simulink model "ForwardKinematic_YuMi"  (R2024a)
(part 13 of 23)

(7514214926474921*sin(q2L)*((4872700232219253*cos(q1L))/9007199254740992 + (6283307137322267*sin(q1L))/9007199254740992))/36893488147419103232))/1152921504606846976 - (67682029681889335677290557259385*cos(q3L)*((7514214926474921*cos(q2L)*((4872700232219253*cos(q1L))/9007199254740992 + (6283307137322267*sin(q1L))/9007199254740992))/36893488147419103232 - sin(q2L)*((6283307137322267*cos(q1L))/9007199254740992 - (4872700232219253*sin(q1L))/9007199254740992)))/332306998946228968225951765070086144))/9007199254740992 - (7514214926474921*sin(q5L)*(((234819211581865*cos(q4L))/1152921504606846976 + (9007199067919185*sin(q4L))/9007199254740992)*((329794241748012540206902858004467560228111939405*cos(q1L))/2993155353253689176481146537402947624255349848014848 + (425266980168672787164801917791314326747055225795*sin(q1L))/2993155353253689176481146537402947624255349848014848 - (67682029681889335677290557259385*cos(q2L)*((4872700232219253*cos(q1L))/9007199254740992 + (6283307137322267*sin(q1L))/9007199254740992))/332306998946228968225951765070086144 + (9007199067919185*sin(q2L)*((6283307137322267*cos(q1L))/9007199254740992 - (4872700232219253*sin(q1L))/9007199254740992))/9007199254740992) + ((4503599440548691*cos(q4L))/4503599627370496 - (7514214926474921*sin(q4L))/36893488147419103232)*((7514214926474921*sin(q3L)*((7514214926474921*cos(q2L)*((4872700232219253*cos(q1L))/9007199254740992 + (6283307137322267*sin(q1L))/9007199254740992))/36893488147419103232 - sin(q2L)*((6283307137322267*cos(q1L))/9007199254740992 - (4872700232219253*sin(q1L))/9007199254740992)))/36893488147419103232 + (9007199067919185*sin(q3L)*((43889380989894851923989405068805*cos(q1L))/81129638414606681695789005144064 + (56594998190739085871744456992395*sin(q1L))/81129638414606681695789005144064))/9007199254740992 - cos(q3L)*(cos(q2L)*((6283307137322267*cos(q1L))/9007199254740992 - (4872700232219253*sin(q1L))/9007199254740992) + (7514214926474921*sin(q2L)*((4872700232219253*cos(q1L))/9007199254740992 + (6283307137322267*sin(q1L))/9007199254740992))/36893488147419103232)) + (7514214926474921*cos(q4L)*(sin(q3L)*(cos(q2L)*((6283307137322267*cos(q1L))/9007199254740992 - (4872700232219253*sin(q1L))/9007199254740992) + (7514214926474921*sin(q2L)*((4872700232219253*cos(q1L))/9007199254740992 + (6283307137322267*sin(q1L))/9007199254740992))/36893488147419103232) + (9007199067919185*cos(q3L)*((43889380989894851923989405068805*cos(q1L))/81129638414606681695789005144064 + (56594998190739085871744456992395*sin(q1L))/81129638414606681695789005144064))/9007199254740992 + (7514214926474921*cos(q3L)*((7514214926474921*cos(q2L)*((4872700232219253*cos(q1L))/9007199254740992 + (6283307137322267*sin(q1L))/9007199254740992))/36893488147419103232 - sin(q2L)*((6283307137322267*cos(q1L))/9007199254740992 - (4872700232219253*sin(q1L))/9007199254740992)))/36893488147419103232))/36893488147419103232))/36893488147419103232 + cos(q5L)*(((7514214926474921*cos(q4L))/36893488147419103232 + (4503599440548691*sin(q4L))/4503599627370496)*((7514214926474921*sin(q3L)*((7514214926474921*cos(q2L)*((4872700232219253*cos(q1L))/9007199254740992 + (6283307137322267*sin(q1L))/9007199254740992))/36893488147419103232 - sin(q2L)*((6283307137322267*cos(q1L))/9007199254740992 - (4872700232219253*sin(q1L))/9007199254740992)))/36893488147419103232 + (9007199067919185*sin(q3L)*((43889380989894851923989405068805*cos(q1L))/81129638414606681695789005144064 + (56594998190739085871744456992395*sin(q1L))/81129638414606681695789005144064))/9007199254740992 - cos(q3L)*(cos(q2L)*((6283307137322267*cos(q1L))/9007199254740992 - (4872700232219253*sin(q1L))/9007199254740992) + (7514214926474921*sin(q2L)*((4872700232219253*cos(q1L))/9007199254740992 + (6283307137322267*sin(q1L))/9007199254740992))/36893488147419103232)) - ((9007199067919185*cos(q4L))/9007199254740992 - (234819211581865*sin(q4L))/1152921504606846976)*((329794241748012540206902858004467560228111939405*cos(q1L))/2993155353253689176481146537402947624255349848014848 + (425266980168672787164801917791314326747055225795*sin(q1L))/2993155353253689176481146537402947624255349848014848 - (67682029681889335677290557259385*cos(q2L)*((4872700232219253*cos(q1L))/9007199254740992 + (6283307137322267*sin(q1L))/9007199254740992))/332306998946228968225951765070086144 + (9007199067919185*sin(q2L)*((6283307137322267*cos(q1L))/9007199254740992 - (4872700232219253*sin(q1L))/9007199254740992))/9007199254740992) + (7514214926474921*sin(q4L)*(sin(q3L)*(cos(q2L)*((6283307137322267*cos(q1L))/9007199254740992 - (4872700232219253*sin(q1L))/9007199254740992) + (7514214926474921*sin(q2L)*((4872700232219253*cos(q1L))/9007199254740992 + (6283307137322267*sin(q1L))/9007199254740992))/36893488147419103232) + (9007199067919185*cos(q3L)*((43889380989894851923989405068805*cos(q1L))/81129638414606681695789005144064 + (56594998190739085871744456992395*sin(q1L))/81129638414606681695789005144064))/9007199254740992 + (7514214926474921*cos(q3L)*((7514214926474921*cos(q2L)*((4872700232219253*cos(q1L))/9007199254740992 + (6283307137322267*sin(q1L))/9007199254740992))/36893488147419103232 - sin(q2L)*((6283307137322267*cos(q1L))/9007199254740992 - (4872700232219253*sin(q1L))/9007199254740992)))/36893488147419103232))/36893488147419103232)))/1000 + (202883803014822867*sin(q6L)*((7514214926474921*cos(q5L)*(((234819211581865*cos(q4L))/1152921504606846976 + (9007199067919185*sin(q4L))/9007199254740992)*((329794241748012540206902858004467560228111939405*cos(q1L))/2993155353253689176481146537402947624255349848014848 + (425266980168672787164801917791314326747055225795*sin(q1L))/2993155353253689176481146537402947624255349848014848 - (67682029681889335677290557259385*cos(q2L)*((4872700232219253*cos(q1L))/9007199254740992 + (6283307137322267*sin(q1L))/9007199254740992))/332306998946228968225951765070086144 + (9007199067919185*sin(q2L)*((6283307137322267*cos(q1L))/9007199254740992 - (4872700232219253*sin(q1L))/9007199254740992))/9007199254740992) + ((4503599440548691*cos(q4L))/4503599627370496 - (7514214926474921*sin(q4L))/36893488147419103232)*((7514214926474921*sin(q3L)*((7514214926474921*cos(q2L)*((4872700232219253*cos(q1L))/9007199254740992 + (6283307137322267*sin(q1L))/9007199254740992))/36893488147419103232 - sin(q2L)*((6283307137322267*cos(q1L))/9007199254740992 - (4872700232219253*sin(q1L))/9007199254740992)))/36893488147419103232 + (9007199067919185*sin(q3L)*((43889380989894851923989405068805*cos(q1L))/81129638414606681695789005144064 + (56594998190739085871744456992395*sin(q1L))/81129638414606681695789005144064))/9007199254740992 - cos(q3L)*(cos(q2L)*((6283307137322267*cos(q1L))/9007199254740992 - (4872700232219253*sin(q1L))/9007199254740992) + (7514214926474921*sin(q2L)*((4872700232219253*cos(q1L))/9007199254740992 + (6283307137322267*sin(q1L))/9007199254740992))/36893488147419103232)) + (7514214926474921*cos(q4L)*(sin(q3L)*(cos(q2L)*((6283307137322267*cos(q1L))/9007199254740992 - (4872700232219253*sin(q1L))/9007199254740992) + (7514214926474921*sin(q2L)*((4872700232219253*cos(q1L))/9007199254740992 + (6283307137322267*sin(q1L))/9007199254740992))/36893488147419103232) + (9007199067919185*cos(q3L)*((43889380989894851923989405068805*cos(q1L))/81129638414606681695789005144064 + (56594998190739085871744456992395*sin(q1L))/81129638414606681695789005144064))/9007199254740992 + (7514214926474921*cos(q3L)*((7514214926474921*cos(q2L)*((4872700232219253*cos(q1L))/9007199254740992 + (6283307137322267*sin(q1L))/9007199254740992))/36893488147419103232 - sin(q2L)*((6283307137322267*cos(q1L))/9007199254740992 - (4872700232219253*sin(q1L))/9007199254740992)))/36893488147419103232))/36893488147419103232))/36893488147419103232 - (9007199067919185*cos(q5L)*((516845254133432670685844229576986303733782399690601453662320875*cos(q1L))/113078212145816597093331040047546785012958969400039613319782796882727665664 + (666467732349846997487583938718911583194406904318712922873589125*sin(q1L))/113078212145816597093331040047546785012958969400039613319782796882727665664 - (9007199067919185*sin(q3L)*(cos(q2L)*((6283307137322267*cos(q1L))/9007199254740992 - (4872700232219253*sin(q1L))/9007199254740992) + (7514214926474921*sin(q2L)*((4872700232219253*cos(q1L))/9007199254740992 + (6283307137322267*sin(q1L))/9007199254740992))/36893488147419103232))/9007199254740992 + (1764482024691522628700660907665*sin(q3L)*((7514214926474921*cos(q2L)*((4872700232219253*cos(q1L))/9007199254740992 + (6283307137322267*sin(q1L))/9007199254740992))/36893488147419103232 - sin(q2L)*((6283307137322267*cos(q1L))/9007199254740992 - (4872700232219253*sin(q1L))/9007199254740992)))/42535295865117307932921825928971026432 - (106069577339469832923929692356850887620017617375*cos(q2L)*((4872700232219253*cos(q1L))/9007199254740992 + (6283307137322267*sin(q1L))/9007199254740992))/12554203470773361527671578846415332832204710888928069025792 + (14115856197532180673579726082375*sin(q2L)*((6283307137322267*cos(q1L))/9007199254740992 - (4872700232219253*sin(q1L))/9007199254740992))/340282366920938463463374607431768211456 - (81129635049124235038645691064225*cos(q3L)*((43889380989894851923989405068805*cos(q1L))/81129638414606681695789005144064 + (56594998190739085871744456992395*sin(q1L))/81129638414606681695789005144064))/81129638414606681695789005144064 + (2115063383689692319117831580025*sin(q3L)*((43889380989894851923989405068805*cos(q1L))/81129638414606681695789005144064 + (56594998190739085871744456992395*sin(q1L))/81129638414606681695789005144064))/10384593717069655257060992658440192 - (234819211581865*cos(q3L)*(cos(q2L)*((6283307137322267*cos(q1L))/9007199254740992 - (4872700232219253*sin(q1L))/9007199254740992) + (7514214926474921*sin(q2L)*((4872700232219253*cos(q1L))/9007199254740992 + (6283307137322267*sin(q1L))/9007199254740992))/36893488147419103232))/1152921504606846976 - (67682029681889335677290557259385*cos(q3L)*((7514214926474921*cos(q2L)*((4872700232219253*cos(q1L))/9007199254740992 + (6283307137322267*sin(q1L))/9007199254740992))/36893488147419103232 - sin(q2L)*((6283307137322267*cos(q1L))/9007199254740992 - (4872700232219253*sin(q1L))/9007199254740992)))/332306998946228968225951765070086144))/9007199254740992 + sin(q5L)*(((7514214926474921*cos(q4L))/36893488147419103232 + (4503599440548691*sin(q4L))/4503599627370496)*((7514214926474921*sin(q3L)*((7514214926474921*cos(q2L)*((4872700232219253*cos(q1L))/9007199254740992 + (6283307137322267*sin(q1L))/9007199254740992))/36893488147419103232 - sin(q2L)*((6283307137322267*cos(q1L))/9007199254740992 - (4872700232219253*sin(q1L))/9007199254740992)))/36893488147419103232 + (9007199067919185*sin(q3L)*((43889380989894851923989405068805*cos(q1L))/81129638414606681695789005144064 + (56594998190739085871744456992395*sin(q1L))/81129638414606681695789005144064))/9007199254740992 - cos(q3L)*(cos(q2L)*((6283307137322267*cos(q1L))/9007199254740992 - (4872700232219253*sin(q1L))/9007199254740992) + (7514214926474921*sin(q2L)*((4872700232219253*cos(q1L))/9007199254740992 + (6283307137322267*sin(q1L))/9007199254740992))/36893488147419103232)) - ((9007199067919185*cos(q4L))/9007199254740992 - (234819211581865*sin(q4L))/1152921504606846976)*((329794241748012540206902858004467560228111939405*cos(q1L))/2993155353253689176481146537402947624255349848014848 + (425266980168672787164801917791314326747055225795*sin(q1L))/2993155353253689176481146537402947624255349848014848 - (67682029681889335677290557259385*cos(q2L)*((4872700232219253*cos(q1L))/9007199254740992 + (6283307137322267*sin(q1L))/9007199254740992))/332306998946228968225951765070086144 + (9007199067919185*sin(q2L)*((6283307137322267*cos(q1L))/9007199254740992 - (4872700232219253*sin(q1L))/9007199254740992))/9007199254740992) + (7514214926474921*sin(q4L)*(sin(q3L)*(cos(q2L)*((6283307137322267*cos(q1L))/9007199254740992 - (4872700232219253*sin(q1L))/9007199254740992) + (7514214926474921*sin(q2L)*((4872700232219253*cos(q1L))/9007199254740992 + (6283307137322267*sin(q1L))/9007199254740992))/36893488147419103232) + (9007199067919185*cos(q3L)*((43889380989894851923989405068805*cos(q1L))/81129638414606681695789005144064 + (56594998190739085871744456992395*sin(q1L))/81129638414606681695789005144064))/9007199254740992 + (7514214926474921*cos(q3L)*((7514214926474921*cos(q2L)*((4872700232219253*cos(q1L))/9007199254740992 + (6283307137322267*sin(q1L))/9007199254740992))/36893488147419103232 - sin(q2L)*((6283307137322267*cos(q1L))/9007199254740992 - (4872700232219253*sin(q1L))/9007199254740992)))/36893488147419103232))/36893488147419103232)))/36893488147419103232000 - (22542644779424763*sin(q2L)*((4872700232219253*cos(q1L))/9007199254740992 + (6283307137322267*sin(q1L))/9007199254740992))/3689348814741910323200 - (107465779053290185796889472867275736954369330186921663479979246519176992895505610212310958309481948671*sin(q2L)*((6283307137322267*cos(q1L))/9007199254740992 - (4872700232219253*sin(q1L))/9007199254740992))/427197407184182016479004341233910422920540904471330553989408321564443945156128110004592417387315200000 - (324259171862923063*sin(q6L)*((9007199067919185*sin(q5L)*((516845254133432670685844229576986303733782399690601453662320875*cos(q1L))/113078212145816597093331040047546785012958969400039613319782796882727665664 + (666467732349846997487583938718911583194406904318712922873589125*sin(q1L))/113078212145816597093331040047546785012958969400039613319782796882727665664 - (9007199067919185*sin(q3L)*(cos(q2L)*((6283307137322267*cos(q1L))/9007199254740992 - (4872700232219253*sin(q1L))/9007199254740992) + (7514214926474921*sin(q2L)*((4872700232219253*cos(q1L))/9007199254740992 + (6283307137322267*sin(q1L))/9007199254740992))/36893488147419103232))/9007199254740992 + (1764482024691522628700660907665*sin(q3L)*((7514214926474921*cos(q2L)*((4872700232219253*cos(q1L))/9007199254740992 + (6283307137322267*sin(q1L))/9007199254740992))/36893488147419103232 - sin(q2L)*((6283307137322267*cos(q1L))/9007199254740992 - (4872700232219253*sin(q1L))/9007199254740992)))/42535295865117307932921825928971026432 - (106069577339469832923929692356850887620017617375*cos(q2L)*((4872700232219253*cos(q1L))/9007199254740992 + (6283307137322267*sin(q1L))/9007199254740992))/12554203470773361527671578846415332832204710888928069025792 + (14115856197532180673579726082375*sin(q2L)*((6283307137322267*cos(q1L))/9007199254740992 - (4872700232219253*sin(q1L))/9007199254740992))/340282366920938463463374607431768211456 - (81129635049124235038645691064225*cos(q3L)*((43889380989894851923989405068805*cos(q1L))/81129638414606681695789005144064 + (56594998190739085871744456992395*sin(q1L))/81129638414606681695789005144064))/81129638414606681695789005144064 + (2115063383689692319117831580025*sin(q3L)*((43889380989894851923989405068805*cos(q1L))/81129638414606681695789005144064 + (56594998190739085871744456992395*sin(q1L))/81129638414606681695789005144064))/10384593717069655257060992658440192 - (234819211581865*cos(q3L)*(cos(q2L)*((6283307137322267*cos(q1L))/9007199254740992 - (4872700232219253*sin(q1L))/9007199254740992) + (7514214926474921*sin(q2L)*((4872700232219253*cos(q1L))/9007199254740992 + (6283307137322267*sin(q1L))/9007199254740992))/36893488147419103232))/1152921504606846976 - (67682029681889335677290557259385*cos(q3L)*((7514214926474921*cos(q2L)*((4872700232219253*cos(q1L))/9007199254740992 + (6283307137322267*sin(q1L))/9007199254740992))/36893488147419103232 - sin(q2L)*((6283307137322267*cos(q1L))/9007199254740992 - (4872700232219253*sin(q1L))/9007199254740992)))/332306998946228968225951765070086144))/9007199254740992 - (7514214926474921*sin(q5L)*(((234819211581865*cos(q4L))/1152921504606846976 + (9007199067919185*sin(q4L))/9007199254740992)*((329794241748012540206902858004467560228111939405*cos(q1L))/2993155353253689176481146537402947624255349848014848 + (425266980168672787164801917791314326747055225795*sin(q1L))/2993155353253689176481146537402947624255349848014848 - (67682029681889335677290557259385*cos(q2L)*((4872700232219253*cos(q1L))/9007199254740992 + (6283307137322267*sin(q1L))/9007199254740992))/332306998946228968225951765070086144 + (9007199067919185*sin(q2L)*((6283307137322267*cos(q1L))/9007199254740992 - (4872700232219253*sin(q1L))/9007199254740992))/9007199254740992) + ((4503599440548691*cos(q4L))/4503599627370496 - (7514214926474921*sin(q4L))/36893488147419103232)*((7514214926474921*sin(q3L)*((7514214926474921*cos(q2L)*((4872700232219253*cos(q1L))/9007199254740992 + (6283307137322267*sin(q1L))/9007199254740992))/36893488147419103232 - sin(q2L)*((6283307137322267*cos(q1L))/9007199254740992 - (4872700232219253*sin(q1L))/9007199254740992)))/36893488147419103232 + (9007199067919185*sin(q3L)*((43889380989894851923989405068805*cos(q1L))/81129638414606681695789005144064 + (56594998190739085871744456992395*sin(q1L))/81129638414606681695789005144064))/9007199254740992 - cos(q3L)*(cos(q2L)*((6283307137322267*cos(q1L))/9007199254740992 - (4872700232219253*sin(q1L))/9007199254740992) + (7514214926474921*sin(q2L)*((4872700232219253*cos(q1L))/9007199254740992 + (6283307137322267*sin(q1L))/9007199254740992))/36893488147419103232)) + (7514214926474921*cos(q4L)*(sin(q3L)*(cos(q2L)*((6283307137322267*cos(q1L))/9007199254740992 - (4872700232219253*sin(q1L))/9007199254740992) + (7514214926474921*sin(q2L)*((4872700232219253*cos(q1L))/9007199254740992 + (6283307137322267*sin(q1L))/9007199254740992))/36893488147419103232) + (9007199067919185*cos(q3L)*((43889380989894851923989405068805*cos(q1L))/81129638414606681695789005144064 + (56594998190739085871744456992395*sin(q1L))/81129638414606681695789005144064))/9007199254740992 + (7514214926474921*cos(q3L)*((7514214926474921*cos(q2L)*((4872700232219253*cos(q1L))/9007199254740992 + (6283307137322267*sin(q1L))/9007199254740992))/36893488147419103232 - sin(q2L)*((6283307137322267*cos(q1L))/9007199254740992 - (4872700232219253*sin(q1L))/9007199254740992)))/36893488147419103232))/36893488147419103232))/36893488147419103232 + cos(q5L)*(((7514214926474921*cos(q4L))/36893488147419103232 + (4503599440548691*sin(q4L))/4503599627370496)*((7514214926474921*sin(q3L)*((7514214926474921*cos(q2L)*((4872700232219253*cos(q1L))/9007199254740992 + (6283307137322267*sin(q1L))/9007199254740992))/36893488147419103232 - sin(q2L)*((6283307137322267*cos(q1L))/9007199254740992 - (4872700232219253*sin(q1L))/9007199254740992)))/36893488147419103232 + (9007199067919185*sin(q3L)*((43889380989894851923989405068805*cos(q1L))/81129638414606681695789005144064 + (56594998190739085871744456992395*sin(q1L))/81129638414606681695789005144064))/9007199254740992 - cos(q3L)*(cos(q2L)*((6283307137322267*cos(q1L))/9007199254740992 - (4872700232219253*sin(q1L))/9007199254740992) + (7514214926474921*sin(q2L)*((4872700232219253*cos(q1L))/9007199254740992 + (6283307137322267*sin(q1L))/9007199254740992))/36893488147419103232)) - ((9007199067919185*cos(q4L))/9007199254740992 - (234819211581865*sin(q4L))/1152921504606846976)*((329794241748012540206902858004467560228111939405*cos(q1L))/2993155353253689176481146537402947624255349848014848 + (425266980168672787164801917791314326747055225795*sin(q1L))/2993155353253689176481146537402947624255349848014848 - (67682029681889335677290557259385*cos(q2L)*((4872700232219253*cos(q1L))/9007199254740992 + (6283307137322267*sin(q1L))/9007199254740992))/332306998946228968225951765070086144 + (9007199067919185*sin(q2L)*((6283307137322267*cos(q1L))/9007199254740992 - (4872700232219253*sin(q1L))/9007199254740992))/9007199254740992) + (7514214926474921*sin(q4L)*(sin(q3L)*(cos(q2L)*((6283307137322267*cos(q1L))/9007199254740992 - (4872700232219253*sin(q1L))/9007199254740992) + (7514214926474921*sin(q2L)*((4872700232219253*cos(q1L))/9007199254740992 + (6283307137322267*sin(q1L))/9007199254740992))/36893488147419103232) + (9007199067919185*cos(q3L)*((43889380989894851923989405068805*cos(q1L))/81129638414606681695789005144064 + (56594998190739085871744456992395*sin(q1L))/81129638414606681695789005144064))/9007199254740992 + (7514214926474921*cos(q3L)*((7514214926474921*cos(q2L)*((4872700232219253*cos(q1L))/9007199254740992 + (6283307137322267*sin(q1L))/9007199254740992))/36893488147419103232 - sin(q2L)*((6283307137322267*cos(q1L))/9007199254740992 - (4872700232219253*sin(q1L))/9007199254740992)))/36893488147419103232))/36893488147419103232)))/9007199254740992000 - (712008244765680093343103025701132101054572137019*cos(q5L)*(((234819211581865*cos(q4L))/1152921504606846976 + (9007199067919185*sin(q4L))/9007199254740992)*((329794241748012540206902858004467560228111939405*cos(q1L))/2993155353253689176481146537402947624255349848014848 + (425266980168672787164801917791314326747055225795*sin(q1L))/2993155353253689176481146537402947624255349848014848 - (67682029681889335677290557259385*cos(q2L)*((4872700232219253*cos(q1L))/9007199254740992 + (6283307137322267*sin(q1L))/9007199254740992))/332306998946228968225951765070086144 + (9007199067919185*sin(q2L)*((6283307137322267*cos(q1L))/9007199254740992 - (4872700232219253*sin(q1L))/9007199254740992))/9007199254740992) + ((4503599440548691*cos(q4L))/4503599627370496 - (7514214926474921*sin(q4L))/36893488147419103232)*((7514214926474921*sin(q3L)*((7514214926474921*cos(q2L)*((4872700232219253*cos(q1L))/9007199254740992 + (6283307137322267*sin(q1L))/9007199254740992))/36893488147419103232 - sin(q2L)*((6283307137322267*cos(q1L))/9007199254740992 - (4872700232219253*sin(q1L))/9007199254740992)))/36893488147419103232 + (9007199067919185*sin(q3L)*((43889380989894851923989405068805*cos(q1L))/81129638414606681695789005144064 + (56594998190739085871744456992395*sin(q1L))/81129638414606681695789005144064))/9007199254740992 - cos(q3L)*(cos(q2L)*((6283307137322267*cos(q1L))/9007199254740992 - (4872700232219253*sin(q1L))/9007199254740992) + (7514214926474921*sin(q2L)*((4872700232219253*cos(q1L))/9007199254740992 + (6283307137322267*sin(q1L))/9007199254740992))/36893488147419103232)) + (7514214926474921*cos(q4L)*(sin(q3L)*(cos(q2L)*((6283307137322267*cos(q1L))/9007199254740992 - (4872700232219253*sin(q1L))/9007199254740992) + (7514214926474921*sin(q2L)*((4872700232219253*cos(q1L))/9007199254740992 + (6283307137322267*sin(q1L))/9007199254740992))/36893488147419103232) + (9007199067919185*cos(q3L)*((43889380989894851923989405068805*cos(q1L))/81129638414606681695789005144064 + (56594998190739085871744456992395*sin(q1L))/81129638414606681695789005144064))/9007199254740992 + (7514214926474921*cos(q3L)*((7514214926474921*cos(q2L)*((4872700232219253*cos(q1L))/9007199254740992 + (6283307137322267*sin(q1L))/9007199254740992))/36893488147419103232 - sin(q2L)*((6283307137322267*cos(q1L))/9007199254740992 - (4872700232219253*sin(q1L))/9007199254740992)))/36893488147419103232))/36893488147419103232))/2451992865385422173373355243440494693789982595493763481600 + (202883803014822867*sin(q5L)*(((234819211581865*cos(q4L))/1152921504606846976 + (9007199067919185*sin(q4L))/9007199254740992)*((329794241748012540206902858004467560228111939405*cos(q1L))/2993155353253689176481146537402947624255349848014848 + (425266980168672787164801917791314326747055225795*sin(q1L))/2993155353253689176481146537402947624255349848014848 - (67682029681889335677290557259385*cos(q2L)*((4872700232219253*cos(q1L))/9007199254740992 + (6283307137322267*sin(q1L))/9007199254740992))/332306998946228968225951765070086144 + (9007199067919185*sin(q2L)*((6283307137322267*cos(q1L))/9007199254740992 - (4872700232219253*sin(q1L))/9007199254740992))/9007199254740992) + ((4503599440548691*cos(q4L))/4503599627370496 - (7514214926474921*sin(q4L))/36893488147419103232)*((7514214926474921*sin(q3L)*((7514214926474921*cos(q2L)*((4872700232219253*cos(q1L))/9007199254740992 + (6283307137322267*sin(q1L))/9007199254740992))/36893488147419103232 - sin(q2L)*((6283307137322267*cos(q1L))/9007199254740992 - (4872700232219253*sin(q1L))/9007199254740992)))/36893488147419103232 + (9007199067919185*sin(q3L)*((43889380989894851923989405068805*cos(q1L))/81129638414606681695789005144064 + (56594998190739085871744456992395*sin(q1L))/81129638414606681695789005144064))/9007199254740992 - cos(q3L)*(cos(q2L)*((6283307137322267*cos(q1L))/9007199254740992 - (4872700232219253*sin(q1L))/9007199254740992) + (7514214926474921*sin(q2L)*((4872700232219253*cos(q1L))/9007199254740992 + (6283307137322267*sin(q1L))/9007199254740992))/36893488147419103232)) + (7514214926474921*cos(q4L)*(sin(q3L)*(cos(q2L)*((6283307137322267*cos(q1L))/9007199254740992 - (4872700232219253*sin(q1L))/9007199254740992) + (7514214926474921*sin(q2L)*((4872700232219253*cos(q1L))/9007199254740992 + (6283307137322267*sin(q1L))/9007199254740992))/36893488147419103232) + (9007199067919185*cos(q3L)*((43889380989894851923989405068805*cos(q1L))/81129638414606681695789005144064 + (56594998190739085871744456992395*sin(q1L))/81129638414606681695789005144064))/9007199254740992 + (7514214926474921*cos(q3L)*((7514214926474921*cos(q2L)*((4872700232219253*cos(q1L))/9007199254740992 + (6283307137322267*sin(q1L))/9007199254740992))/36893488147419103232 - sin(q2L)*((6283307137322267*cos(q1L))/9007199254740992 - (4872700232219253*sin(q1L))/9007199254740992)))/36893488147419103232))/36893488147419103232))/36893488147419103232000 - (27*cos(q5L)*(((7514214926474921*cos(q4L))/36893488147419103232 + (4503599440548691*sin(q4L))/4503599627370496)*((7514214926474921*sin(q3L)*((7514214926474921*cos(q2L)*((4872700232219253*cos(q1L))/9007199254740992 + (6283307137322267*sin(q1L))/9007199254740992))/36893488147419103232 - sin(q2L)*((6283307137322267*cos(q1L))/9007199254740992 - (4872700232219253*sin(q1L))/9007199254740992)))/36893488147419103232 + (9007199067919185*sin(q3L)*((43889380989894851923989405068805*cos(q1L))/81129638414606681695789005144064 + (56594998190739085871744456992395*sin(q1L))/81129638414606681695789005144064))/9007199254740992 - cos(q3L)*(cos(q2L)*((6283307137322267*cos(q1L))/9007199254740992 - (4872700232219253*sin(q1L))/9007199254740992) + (7514214926474921*sin(q2L)*((4872700232219253*cos(q1L))/9007199254740992 + (6283307137322267*sin(q1L))/9007199254740992))/36893488147419103232)) - ((9007199067919185*cos(q4L))/9007199254740992 - (234819211581865*sin(q4L))/1152921504606846976)*((329794241748012540206902858004467560228111939405*cos(q1L))/2993155353253689176481146537402947624255349848014848 + (425266980168672787164801917791314326747055225795*sin(q1L))/2993155353253689176481146537402947624255349848014848 - (67682029681889335677290557259385*cos(q2L)*((4872700232219253*cos(q1L))/9007199254740992 + (6283307137322267*sin(q1L))/9007199254740992))/332306998946228968225951765070086144 + (9007199067919185*sin(q2L)*((6283307137322267*cos(q1L))/9007199254740992 - (4872700232219253*sin(q1L))/9007199254740992))/9007199254740992) + (7514214926474921*sin(q4L)*(sin(q3L)*(cos(q2L)*((6283307137322267*cos(q1L))/9007199254740992 - (4872700232219253*sin(q1L))/9007199254740992) + (7514214926474921*sin(q2L)*((4872700232219253*cos(q1L))/9007199254740992 + (6283307137322267*sin(q1L))/9007199254740992))/36893488147419103232) + (9007199067919185*cos(q3L)*((43889380989894851923989405068805*cos(q1L))/81129638414606681695789005144064 + (56594998190739085871744456992395*sin(q1L))/81129638414606681695789005144064))/9007199254740992 + (7514214926474921*cos(q3L)*((7514214926474921*cos(q2L)*((4872700232219253*cos(q1L))/9007199254740992 + (6283307137322267*sin(q1L))/9007199254740992))/36893488147419103232 - sin(q2L)*((6283307137322267*cos(q1L))/9007199254740992 - (4872700232219253*sin(q1L))/9007199254740992)))/36893488147419103232))/36893488147419103232))/1000 - (94754841554645069948206780163139*sin(q5L)*(((7514214926474921*cos(q4L))/36893488147419103232 + (4503599440548691*sin(q4L))/4503599627370496)*((7514214926474921*sin(q3L)*((7514214926474921*cos(q2L)*((4872700232219253*cos(q1L))/9007199254740992 + (6283307137322267*sin(q1L))/9007199254740992))/36893488147419103232 - sin(q2L)*((6283307137322267*cos(q1L))/9007199254740992 - (4872700232219253*sin(q1L))/9007199254740992)))/36893488147419103232 + (9007199067919185*sin(q3L)*((43889380989894851923989405068805*cos(q1L))/81129638414606681695789005144064 + (56594998190739085871744456992395*sin(q1L))/81129638414606681695789005144064))/9007199254740992 - cos(q3L)*(cos(q2L)*((6283307137322267*cos(q1L))/9007199254740992 - (4872700232219253*sin(q1L))/9007199254740992) + (7514214926474921*sin(q2L)*((4872700232219253*cos(q1L))/9007199254740992 + (6283307137322267*sin(q1L))/9007199254740992))/36893488147419103232)) - ((9007199067919185*cos(q4L))/9007199254740992 - (234819211581865*sin(q4L))/1152921504606846976)*((329794241748012540206902858004467560228111939405*cos(q1L))/2993155353253689176481146537402947624255349848014848 + (425266980168672787164801917791314326747055225795*sin(q1L))/2993155353253689176481146537402947624255349848014848 - (67682029681889335677290557259385*cos(q2L)*((4872700232219253*cos(q1L))/9007199254740992 + (6283307137322267*sin(q1L))/9007199254740992))/332306998946228968225951765070086144 + (9007199067919185*sin(q2L)*((6283307137322267*cos(q1L))/9007199254740992 - (4872700232219253*sin(q1L))/9007199254740992))/9007199254740992) + (7514214926474921*sin(q4L)*(sin(q3L)*(cos(q2L)*((6283307137322267*cos(q1L))/9007199254740992 - (4872700232219253*sin(q1L))/9007199254740992) + (7514214926474921*sin(q2L)*((4872700232219253*cos(q1L))/9007199254740992 + (6283307137322267*sin(q1L))/9007199254740992))/36893488147419103232) + (9007199067919185*cos(q3L)*((43889380989894851923989405068805*cos(q1L))/81129638414606681695789005144064 + (56594998190739085871744456992395*sin(q1L))/81129638414606681695789005144064))/9007199254740992 + (7514214926474921*cos(q3L)*((7514214926474921*cos(q2L)*((4872700232219253*cos(q1L))/9007199254740992 + (6283307137322267*sin(q1L))/9007199254740992))/36893488147419103232 - sin(q2L)*((6283307137322267*cos(q1L))/9007199254740992 - (4872700232219253*sin(q1L))/9007199254740992)))/36893488147419103232))/36893488147419103232))/66461399789245793645190353014017228800 - (83301539375654672537075965313343183841442266989297270401707771044036658496661398777306991*cos(q3L)*((43889380989894851923989405068805*cos(q1L))/81129638414606681695789005144064 + (56594998190739085871744456992395*sin(q1L))/81129638414606681695789005144064))/4074071952668972172536891376818756322102936787331872501272280898708762599526673412366794752000 + (610321541873521657855151997354401418608858870661075444886782706002880706727*cos(q4L)*(sin(q3L)*(cos(q2L)*((6283307137322267*cos(q1L))/9007199254740992 - (4872700232219253*sin(q1L))/9007199254740992) + (7514214926474921*sin(q2L)*((4872700232219253*cos(q1L))/9007199254740992 + (6283307137322267*sin(q1L))/9007199254740992))/36893488147419103232) + (9007199067919185*cos(q3L)*((43889380989894851923989405068805*cos(q1L))/81129638414606681695789005144064 + (56594998190739085871744456992395*sin(q1L))/81129638414606681695789005144064))/9007199254740992 + (7514214926474921*cos(q3L)*((7514214926474921*cos(q2L)*((4872700232219253*cos(q1L))/9007199254740992 + (6283307137322267*sin(q1L))/9007199254740992))/36893488147419103232 - sin(q2L)*((6283307137322267*cos(q1L))/9007199254740992 - (4872700232219253*sin(q1L))/9007199254740992)))/36893488147419103232))/11307821214581659709333104004754678501295896940003961331978279688272766566400000 + (109198173955282063961996941994332957526645881091499469714283881779231664456243735535448036415347*sin(q3L)*((43889380989894851923989405068805*cos(q1L))/81129638414606681695789005144064 + (56594998190739085871744456992395*sin(q1L))/81129638414606681695789005144064))/2607406049708142190423610481164004046145879543892398400814259775173608063697070983914748641280000 + (608651409044468601*sin(q4L)*(sin(q3L)*(cos(q2L)*((6283307137322267*cos(q1L))/9007199254740992 - (4872700232219253*sin(q1L))/9007199254740992) + (7514214926474921*sin(q2L)*((4872700232219253*cos(q1L))/9007199254740992 + (6283307137322267*sin(q1L))/9007199254740992))/36893488147419103232) + (9007199067919185*cos(q3L)*((43889380989894851923989405068805*cos(q1L))/81129638414606681695789005144064 + (56594998190739085871744456992395*sin(q1L))/81129638414606681695789005144064))/9007199254740992 + (7514214926474921*cos(q3L)*((7514214926474921*cos(q2L)*((4872700232219253*cos(q1L))/9007199254740992 + (6283307137322267*sin(q1L))/9007199254740992))/36893488147419103232 - sin(q2L)*((6283307137322267*cos(q1L))/9007199254740992 - (4872700232219253*sin(q1L))/9007199254740992)))/36893488147419103232))/73786976294838206464000 - (60617164743372705924380750591060836759586313939367162716784907429017787816377231*cos(q3L)*(cos(q2L)*((6283307137322267*cos(q1L))/9007199254740992 - (4872700232219253*sin(q1L))/9007199254740992) + (7514214926474921*sin(q2L)*((4872700232219253*cos(q1L))/9007199254740992 + (6283307137322267*sin(q1L))/9007199254740992))/36893488147419103232))/1447401115466452442794637312608598848165874808320507050493219800098914120499200000 - (347469655025336708709976918716104493695816557877713443586884917071777956519687017125887603*cos(q3L)*((7514214926474921*cos(q2L)*((4872700232219253*cos(q1L))/9007199254740992 + (6283307137322267*sin(q1L))/9007199254740992))/36893488147419103232 - sin(q2L)*((6283307137322267*cos(q1L))/9007199254740992 - (4872700232219253*sin(q1L))/9007199254740992)))/83436993590660550093555535397248129476668145404556748826056312805555458038306271485271956520960000, (324259171862923063*sin(q6L)*((7514214926474921*sin(q5L)*(((4503599440548691*cos(q4L))/4503599627370496 - (7514214926474921*sin(q4L))/36893488147419103232)*(cos(q3L)*((7514214926474921*cos(q2L)*((6283307137322267*cos(q1L))/9007199254740992 - (4872700232219253*sin(q1L))/9007199254740992))/36893488147419103232 - (76229820211215127867025072518845*cos(q2L))/162259276829213363391578010288128 + sin(q2L)*((4872700232219253*cos(q1L))/9007199254740992 + (6283307137322267*sin(q1L))/9007199254740992)) - (7514214926474921*sin(q3L)*((76229820211215127867025072518845*sin(q2L))/162259276829213363391578010288128 + cos(q2L)*((4872700232219253*cos(q1L))/9007199254740992 + (6283307137322267*sin(q1L))/9007199254740992) - (7514214926474921*sin(q2L)*((6283307137322267*cos(q1L))/9007199254740992 - (4872700232219253*sin(q1L))/9007199254740992))/36893488147419103232))/36893488147419103232) + ((234819211581865*cos(q4L))/1152921504606846976 + (9007199067919185*sin(q4L))/9007199254740992)*((686617165554103949950999710565799465200849541325*sin(q2L))/1461501637330902918203684832716283019655932542976 + (9007199067919185*cos(q2L)*((4872700232219253*cos(q1L))/9007199254740992 + (6283307137322267*sin(q1L))/9007199254740992))/9007199254740992 - (67682029681889335677290557259385*sin(q2L)*((6283307137322267*cos(q1L))/9007199254740992 - (4872700232219253*sin(q1L))/9007199254740992))/332306998946228968225951765070086144) - (7514214926474921*cos(q4L)*((7514214926474921*cos(q3L)*((76229820211215127867025072518845*sin(q2L))/162259276829213363391578010288128 + cos(q2L)*((4872700232219253*cos(q1L))/9007199254740992 + (6283307137322267*sin(q1L))/9007199254740992) - (7514214926474921*sin(q2L)*((6283307137322267*cos(q1L))/9007199254740992 - (4872700232219253*sin(q1L))/9007199254740992))/36893488147419103232))/36893488147419103232 + sin(q3L)*((7514214926474921*cos(q2L)*((6283307137322267*cos(q1L))/9007199254740992 - (4872700232219253*sin(q1L))/9007199254740992))/36893488147419103232 - (76229820211215127867025072518845*cos(q2L))/162259276829213363391578010288128 + sin(q2L)*((4872700232219253*cos(q1L))/9007199254740992 + (6283307137322267*sin(q1L))/9007199254740992))))/36893488147419103232))/36893488147419103232 + cos(q5L)*(((9007199067919185*cos(q4L))/9007199254740992 - (234819211581865*sin(q4L))/1152921504606846976)*((686617165554103949950999710565799465200849541325*sin(q2L))/1461501637330902918203684832716283019655932542976 + (9007199067919185*cos(q2L)*((4872700232219253*cos(q1L))/9007199254740992 + (6283307137322267*sin(q1L))/9007199254740992))/9007199254740992 - (67682029681889335677290557259385*sin(q2L)*((6283307137322267*cos(q1L))/9007199254740992 - (4872700232219253*sin(q1L))/9007199254740992))/332306998946228968225951765070086144) - ((7514214926474921*cos(q4L))/36893488147419103232 + (4503599440548691*sin(q4L))/4503599627370496)*(cos(q3L)*((7514214926474921*cos(q2L)*((6283307137322267*cos(q1L))/9007199254740992 - (4872700232219253*sin(q1L))/9007199254740992))/36893488147419103232 - (76229820211215127867025072518845*cos(q2L))/162259276829213363391578010288128 + sin(q2L)*((4872700232219253*cos(q1L))/9007199254740992 + (6283307137322267*sin(q1L))/9007199254740992)) - (7514214926474921*sin(q3L)*((76229820211215127867025072518845*sin(q2L))/162259276829213363391578010288128 + cos(q2L)*((4872700232219253*cos(q1L))/9007199254740992 + (6283307137322267*sin(q1L))/9007199254740992) - (7514214926474921*sin(q2L)*((6283307137322267*cos(q1L))/9007199254740992 - (4872700232219253*sin(q1L))/9007199254740992))/36893488147419103232))/36893488147419103232) + (7514214926474921*sin(q4L)*((7514214926474921*cos(q3L)*((76229820211215127867025072518845*sin(q2L))/162259276829213363391578010288128 + cos(q2L)*((4872700232219253*cos(q1L))/9007199254740992 + (6283307137322267*sin(q1L))/9007199254740992) - (7514214926474921*sin(q2L)*((6283307137322267*cos(q1L))/9007199254740992 - (4872700232219253*sin(q1L))/9007199254740992))/36893488147419103232))/36893488147419103232 + sin(q3L)*((7514214926474921*cos(q2L)*((6283307137322267*cos(q1L))/9007199254740992 - (4872700232219253*sin(q1L))/9007199254740992))/36893488147419103232 - (76229820211215127867025072518845*cos(q2L))/162259276829213363391578010288128 + sin(q2L)*((4872700232219253*cos(q1L))/9007199254740992 + (6283307137322267*sin(q1L))/9007199254740992))))/36893488147419103232) - (9007199067919185*sin(q5L)*((1076049180065244948668759145796765391250102872519935285209856875*sin(q2L))/55213970774324510299478046898216203619608871777363092441300193790394368 + (234819211581865*cos(q3L)*((7514214926474921*cos(q2L)*((6283307137322267*cos(q1L))/9007199254740992 - (4872700232219253*sin(q1L))/9007199254740992))/36893488147419103232 - (76229820211215127867025072518845*cos(q2L))/162259276829213363391578010288128 + sin(q2L)*((4872700232219253*cos(q1L))/9007199254740992 + (6283307137322267*sin(q1L))/9007199254740992)))/1152921504606846976 + (67682029681889335677290557259385*cos(q3L)*((76229820211215127867025072518845*sin(q2L))/162259276829213363391578010288128 + cos(q2L)*((4872700232219253*cos(q1L))/9007199254740992 + (6283307137322267*sin(q1L))/9007199254740992) - (7514214926474921*sin(q2L)*((6283307137322267*cos(q1L))/9007199254740992 - (4872700232219253*sin(q1L))/9007199254740992))/36893488147419103232))/332306998946228968225951765070086144 + (9007199067919185*sin(q3L)*((7514214926474921*cos(q2L)*((6283307137322267*cos(q1L))/9007199254740992 - (4872700232219253*sin(q1L))/9007199254740992))/36893488147419103232 - (76229820211215127867025072518845*cos(q2L))/162259276829213363391578010288128 + sin(q2L)*((4872700232219253*cos(q1L))/9007199254740992 + (6283307137322267*sin(q1L))/9007199254740992)))/9007199254740992 - (1764482024691522628700660907665*sin(q3L)*((76229820211215127867025072518845*sin(q2L))/162259276829213363391578010288128 + cos(q2L)*((4872700232219253*cos(q1L))/9007199254740992 + (6283307137322267*sin(q1L))/9007199254740992) - (7514214926474921*sin(q2L)*((6283307137322267*cos(q1L))/9007199254740992 - (4872700232219253*sin(q1L))/9007199254740992))/36893488147419103232))/42535295865117307932921825928971026432 + (14115856197532180673579726082375*cos(q2L)*((4872700232219253*cos(q1L))/9007199254740992 + (6283307137322267*sin(q1L))/9007199254740992))/340282366920938463463374607431768211456 - (106069577339469832923929692356850887620017617375*sin(q2L)*((6283307137322267*cos(q1L))/9007199254740992 - (4872700232219253*sin(q1L))/9007199254740992))/12554203470773361527671578846415332832204710888928069025792))/9007199254740992))/9007199254740992000 - (1638419403218095907026718462896803369073888043416845373610358683372970217080019045088391026475339262573991311605362042051448194040999*sin(q2L))/13863348470604074297892070920715418517182185376879082875852397903073106539028128115199872030520697890486956054807017859144870789120000 - (45737892126729076720215043511307*cos(q2L))/3245185536584267267831560205762560 + (81222263116692158804177042061221826384594597321566869716687*((4503599440548691*cos(q4L))/4503599627370496 - (7514214926474921*sin(q4L))/36893488147419103232)*(cos(q3L)*((7514214926474921*cos(q2L)*((6283307137322267*cos(q1L))/9007199254740992 - (4872700232219253*sin(q1L))/9007199254740992))/36893488147419103232 - (76229820211215127867025072518845*cos(q2L))/162259276829213363391578010288128 + sin(q2L)*((4872700232219253*cos(q1L))/9007199254740992 + (6283307137322267*sin(q1L))/9007199254740992)) - (7514214926474921*sin(q3L)*((76229820211215127867025072518845*sin(q2L))/162259276829213363391578010288128 + cos(q2L)*((4872700232219253*cos(q1L))/9007199254740992 + (6283307137322267*sin(q1L))/9007199254740992) - (7514214926474921*sin(q2L)*((6283307137322267*cos(q1L))/9007199254740992 - (4872700232219253*sin(q1L))/9007199254740992))/36893488147419103232))/36893488147419103232))/306499108173177771671669405430061836723747824436720435200000 + (81*((7514214926474921*cos(q4L))/36893488147419103232 + (4503599440548691*sin(q4L))/4503599627370496)*(cos(q3L)*((7514214926474921*cos(q2L)*((6283307137322267*cos(q1L))/9007199254740992 - (4872700232219253*sin(q1L))/9007199254740992))/36893488147419103232 - (76229820211215127867025072518845*cos(q2L))/162259276829213363391578010288128 + sin(q2L)*((4872700232219253*cos(q1L))/9007199254740992 + (6283307137322267*sin(q1L))/9007199254740992)) - (7514214926474921*sin(q3L)*((76229820211215127867025072518845*sin(q2L))/162259276829213363391578010288128 + cos(q2L)*((4872700232219253*cos(q1L))/9007199254740992 + (6283307137322267*sin(q1L))/9007199254740992) - (7514214926474921*sin(q2L)*((6283307137322267*cos(q1L))/9007199254740992 - (4872700232219253*sin(q1L))/9007199254740992))/36893488147419103232))/36893488147419103232))/2000 + (60617164743372705924380750591060836759586313939367162716784907429017787816377231*cos(q3L)*((7514214926474921*cos(q2L)*((6283307137322267*cos(q1L))/9007199254740992 - (4872700232219253*sin(q1L))/9007199254740992))/36893488147419103232 - (76229820211215127867025072518845*cos(q2L))/162259276829213363391578010288128 + sin(q2L)*((4872700232219253*cos(q1L))/9007199254740992 + (6283307137322267*sin(q1L))/9007199254740992)))/1447401115466452442794637312608598848165874808320507050493219800098914120499200000 + (347469655025336708709976918716104493695816557877713443586884917071777956519687017125887603*cos(q3L)*((76229820211215127867025072518845*sin(q2L))/162259276829213363391578010288128 + cos(q2L)*((4872700232219253*cos(q1L))/9007199254740992 + (6283307137322267*sin(q1L))/9007199254740992) - (7514214926474921*sin(q2L)*((6283307137322267*cos(q1L))/9007199254740992 - (4872700232219253*sin(q1L))/9007199254740992))/36893488147419103232))/83436993590660550093555535397248129476668145404556748826056312805555458038306271485271956520960000 + (46241644459901303158631016767207157814229090534989303509431886332469146043*sin(q3L)*((7514214926474921*cos(q2L)*((6283307137322267*cos(q1L))/9007199254740992 - (4872700232219253*sin(q1L))/9007199254740992))/36893488147419103232 - (76229820211215127867025072518845*cos(q2L))/162259276829213363391578010288128 + sin(q2L)*((4872700232219253*cos(q1L))/9007199254740992 + (6283307137322267*sin(q1L))/9007199254740992)))/2261564242916331941866620800950935700259179388000792266395655937654553313280000 - (455490404115240510935077772268745492204390157443214084883134054419271951750419293234291596923751*sin(q3L)*((76229820211215127867025072518845*sin(q2L))/162259276829213363391578010288128 + cos(q2L)*((4872700232219253*cos(q1L))/9007199254740992 + (6283307137322267*sin(q1L))/9007199254740992) - (7514214926474921*sin(q2L)*((6283307137322267*cos(q1L))/9007199254740992 - (4872700232219253*sin(q1L))/9007199254740992))/36893488147419103232))/53399675898022752059875542654238802865067613058916319248676040195555493144516013750574052173414400000 + (584133382113593486367040631332731*cos(q6L)*((8085664810467363599778659999511780427732698420102663058998013758035866686931875*sin(q2L))/2037035976334486086268445688409378161051468393665936250636140449354381299763336706183397376 + (9007199067919185*((4503599440548691*cos(q4L))/4503599627370496 - (7514214926474921*sin(q4L))/36893488147419103232)*(cos(q3L)*((7514214926474921*cos(q2L)*((6283307137322267*cos(q1L))/9007199254740992 - (4872700232219253*sin(q1L))/9007199254740992))/36893488147419103232 - (76229820211215127867025072518845*cos(q2L))/162259276829213363391578010288128 + sin(q2L)*((4872700232219253*cos(q1L))/9007199254740992 + (6283307137322267*sin(q1L))/9007199254740992)) - (7514214926474921*sin(q3L)*((76229820211215127867025072518845*sin(q2L))/162259276829213363391578010288128 + cos(q2L)*((4872700232219253*cos(q1L))/9007199254740992 + (6283307137322267*sin(q1L))/9007199254740992) - (7514214926474921*sin(q2L)*((6283307137322267*cos(q1L))/9007199254740992 - (4872700232219253*sin(q1L))/9007199254740992))/36893488147419103232))/36893488147419103232))/9007199254740992 + (1764482024691522628700660907665*cos(q3L)*((7514214926474921*cos(q2L)*((6283307137322267*cos(q1L))/9007199254740992 - (4872700232219253*sin(q1L))/9007199254740992))/36893488147419103232 - (76229820211215127867025072518845*cos(q2L))/162259276829213363391578010288128 + sin(q2L)*((4872700232219253*cos(q1L))/9007199254740992 + (6283307137322267*sin(q1L))/9007199254740992)))/42535295865117307932921825928971026432 + (508577317689771495245073589786522929324694383585*cos(q3L)*((76229820211215127867025072518845*sin(q2L))/162259276829213363391578010288128 + cos(q2L)*((4872700232219253*cos(q1L))/9007199254740992 + (6283307137322267*sin(q1L))/9007199254740992) - (7514214926474921*sin(q2L)*((6283307137322267*cos(q1L))/9007199254740992 - (4872700232219253*sin(q1L))/9007199254740992))/36893488147419103232))/12259964326927110866866776217202473468949912977468817408 + (67682029681889335677290557259385*sin(q3L)*((7514214926474921*cos(q2L)*((6283307137322267*cos(q1L))/9007199254740992 - (4872700232219253*sin(q1L))/9007199254740992))/36893488147419103232 - (76229820211215127867025072518845*cos(q2L))/162259276829213363391578010288128 + sin(q2L)*((4872700232219253*cos(q1L))/9007199254740992 + (6283307137322267*sin(q1L))/9007199254740992)))/332306998946228968225951765070086144 - (13258697167433729449897784796786197386719169465*sin(q3L)*((76229820211215127867025072518845*sin(q2L))/162259276829213363391578010288128 + cos(q2L)*((4872700232219253*cos(q1L))/9007199254740992 + (6283307137322267*sin(q1L))/9007199254740992) - (7514214926474921*sin(q2L)*((6283307137322267*cos(q1L))/9007199254740992 - (4872700232219253*sin(q1L))/9007199254740992))/36893488147419103232))/1569275433846670190958947355801916604025588861116008628224 + (106069577339469832923929692356850887620017617375*cos(q2L)*((4872700232219253*cos(q1L))/9007199254740992 + (6283307137322267*sin(q1L))/9007199254740992))/12554203470773361527671578846415332832204710888928069025792 - (797029601289130257223357069404502671534492977261568326111352375*sin(q2L)*((6283307137322267*cos(q1L))/9007199254740992 - (4872700232219253*sin(q1L))/9007199254740992))/463168356949264781694283940034751631413079938662562256157830336031652518559744 + (9007199067919185*((234819211581865*cos(q4L))/1152921504606846976 + (9007199067919185*sin(q4L))/9007199254740992)*((686617165554103949950999710565799465200849541325*sin(q2L))/1461501637330902918203684832716283019655932542976 + (9007199067919185*cos(q2L)*((4872700232219253*cos(q1L))/9007199254740992 + (6283307137322267*sin(q1L))/9007199254740992))/9007199254740992 - (67682029681889335677290557259385*sin(q2L)*((6283307137322267*cos(q1L))/9007199254740992 - (4872700232219253*sin(q1L))/9007199254740992))/332306998946228968225951765070086144))/9007199254740992 - (67682029681889335677290557259385*cos(q4L)*((7514214926474921*cos(q3L)*((76229820211215127867025072518845*sin(q2L))/162259276829213363391578010288128 + cos(q2L)*((4872700232219253*cos(q1L))/9007199254740992 + (6283307137322267*sin(q1L))/9007199254740992) - (7514214926474921*sin(q2L)*((6283307137322267*cos(q1L))/9007199254740992 - (4872700232219253*sin(q1L))/9007199254740992))/36893488147419103232))/36893488147419103232 + sin(q3L)*((7514214926474921*cos(q2L)*((6283307137322267*cos(q1L))/9007199254740992 - (4872700232219253*sin(q1L))/9007199254740992))/36893488147419103232 - (76229820211215127867025072518845*cos(q2L))/162259276829213363391578010288128 + sin(q2L)*((4872700232219253*cos(q1L))/9007199254740992 + (6283307137322267*sin(q1L))/9007199254740992))))/332306998946228968225951765070086144))/16225927682921336339157801028812800 - (107465779053290185796889472867275736954369330186921663479979246519176992895505610212310958309481948671*cos(q2L)*((4872700232219253*cos(q1L))/9007199254740992 + (6283307137322267*sin(q1L))/9007199254740992))/427197407184182016479004341233910422920540904471330553989408321564443945156128110004592417387315200000 + (22542644779424763*cos(q2L)*((6283307137322267*cos(q1L))/9007199254740992 - (4872700232219253*sin(q1L))/9007199254740992))/3689348814741910323200 + (48638874966763599*sin(q6L)*((8085664810467363599778659999511780427732698420102663058998013758035866686931875*sin(q2L))/2037035976334486086268445688409378161051468393665936250636140449354381299763336706183397376 + (9007199067919185*((4503599440548691*cos(q4L))/4503599627370496 - (7514214926474921*sin(q4L))/36893488147419103232)*(cos(q3L)*((7514214926474921*cos(q2L)*((6283307137322267*cos(q1L))/9007199254740992 - (4872700232219253*sin(q1L))/9007199254740992))/36893488147419103232 - (76229820211215127867025072518845*cos(q2L))/162259276829213363391578010288128 + sin(q2L)*((4872700232219253*cos(q1L))/9007199254740992 + (6283307137322267*sin(q1L))/9007199254740992)) - (7514214926474921*sin(q3L)*((76229820211215127867025072518845*sin(q2L))/162259276829213363391578010288128 + cos(q2L)*((4872700232219253*cos(q1L))/9007199254740992 + (6283307137322267*sin(q1L))/9007199254740992) - (7514214926474921*sin(q2L)*((6283307137322267*cos(q1L))/9007199254740992 - (4872700232219253*sin(q1L))/9007199254740992))/36893488147419103232))/36893488147419103232))/9007199254740992 + (1764482024691522628700660907665*cos(q3L)*((7514214926474921*cos(q2L)*((6283307137322267*cos(q1L))/9007199254740992 - (4872700232219253*sin(q1L))/9007199254740992))/36893488147419103232 - (76229820211215127867025072518845*cos(q2L))/162259276829213363391578010288128 + sin(q2L)*((4872700232219253*cos(q1L))/9007199254740992 + (6283307137322267*sin(q1L))/9007199254740992)))/42535295865117307932921825928971026432 + (508577317689771495245073589786522929324694383585*cos(q3L)*((76229820211215127867025072518845*sin(q2L))/162259276829213363391578010288128 + cos(q2L)*((4872700232219253*cos(q1L))/9007199254740992 + (6283307137322267*sin(q1L))/9007199254740992) - (7514214926474921*sin(q2L)*((6283307137322267*cos(q1L))/9007199254740992 - (4872700232219253*sin(q1L))/9007199254740992))/36893488147419103232))/12259964326927110866866776217202473468949912977468817408 + (67682029681889335677290557259385*sin(q3L)*((7514214926474921*cos(q2L)*((6283307137322267*cos(q1L))/9007199254740992 - (4872700232219253*sin(q1L))/9007199254740992))/36893488147419103232 - (76229820211215127867025072518845*cos(q2L))/162259276829213363391578010288128 + sin(q2L)*((4872700232219253*cos(q1L))/9007199254740992 + (6283307137322267*sin(q1L))/9007199254740992)))/332306998946228968225951765070086144 - (13258697167433729449897784796786197386719169465*sin(q3L)*((76229820211215127867025072518845*sin(q2L))/162259276829213363391578010288128 + cos(q2L)*((4872700232219253*cos(q1L))/9007199254740992 + (6283307137322267*sin(q1L))/9007199254740992) - (7514214926474921*sin(q2L)*((6283307137322267*cos(q1L))/9007199254740992 - (4872700232219253*sin(q1L))/9007199254740992))/36893488147419103232))/1569275433846670190958947355801916604025588861116008628224 + (106069577339469832923929692356850887620017617375*cos(q2L)*((4872700232219253*cos(q1L))/9007199254740992 + (6283307137322267*sin(q1L))/9007199254740992))/12554203470773361527671578846415332832204710888928069025792 - (797029601289130257223357069404502671534492977261568326111352375*sin(q2L)*((6283307137322267*cos(q1L))/9007199254740992 - (4872700232219253*sin(q1L))/9007199254740992))/463168356949264781694283940034751631413079938662562256157830336031652518559744 + (9007199067919185*((234819211581865*cos(q4L))/1152921504606846976 + (9007199067919185*sin(q4L))/9007199254740992)*((686617165554103949950999710565799465200849541325*sin(q2L))/1461501637330902918203684832716283019655932542976 + (9007199067919185*cos(q2L)*((4872700232219253*cos(q1L))/9007199254740992 + (6283307137322267*sin(q1L))/9007199254740992))/9007199254740992 - (67682029681889335677290557259385*sin(q2L)*((6283307137322267*cos(q1L))/9007199254740992 - (4872700232219253*sin(q1L))/9007199254740992))/332306998946228968225951765070086144))/9007199254740992 - (67682029681889335677290557259385*cos(q4L)*((7514214926474921*cos(q3L)*((76229820211215127867025072518845*sin(q2L))/162259276829213363391578010288128 + cos(q2L)*((4872700232219253*cos(q1L))/9007199254740992 + (6283307137322267*sin(q1L))/9007199254740992) - (7514214926474921*sin(q2L)*((6283307137322267*cos(q1L))/9007199254740992 - (4872700232219253*sin(q1L))/9007199254740992))/36893488147419103232))/36893488147419103232 + sin(q3L)*((7514214926474921*cos(q2L)*((6283307137322267*cos(q1L))/9007199254740992 - (4872700232219253*sin(q1L))/9007199254740992))/36893488147419103232 - (76229820211215127867025072518845*cos(q2L))/162259276829213363391578010288128 + sin(q2L)*((4872700232219253*cos(q1L))/9007199254740992 + (6283307137322267*sin(q1L))/9007199254740992))))/332306998946228968225951765070086144))/1801439850948198400 - (712008244765680093343103025701132101054572137019*cos(q5L)*(((4503599440548691*cos(q4L))/4503599627370496 - (7514214926474921*sin(q4L))/36893488147419103232)*(cos(q3L)*((7514214926474921*cos(q2L)*((6283307137322267*cos(q1L))/9007199254740992 - (4872700232219253*sin(q1L))/9007199254740992))/36893488147419103232 - (76229820211215127867025072518845*cos(q2L))/162259276829213363391578010288128 + sin(q2L)*((4872700232219253*cos(q1L))/9007199254740992 + (6283307137322267*sin(q1L))/9007199254740992)) - (7514214926474921*sin(q3L)*((76229820211215127867025072518845*sin(q2L))/162259276829213363391578010288128 + cos(q2L)*((4872700232219253*cos(q1L))/9007199254740992 + (6283307137322267*sin(q1L))/9007199254740992) - (7514214926474921*sin(q2L)*((6283307137322267*cos(q1L))/9007199254740992 - (4872700232219253*sin(q1L))/9007199254740992))/36893488147419103232))/36893488147419103232) + ((234819211581865*cos(q4L))/1152921504606846976 + (9007199067919185*sin(q4L))/9007199254740992)*((686617165554103949950999710565799465200849541325*sin(q2L))/1461501637330902918203684832716283019655932542976 + (9007199067919185*cos(q2L)*((4872700232219253*cos(q1L))/9007199254740992 + (6283307137322267*sin(q1L))/9007199254740992))/9007199254740992 - (67682029681889335677290557259385*sin(q2L)*((6283307137322267*cos(q1L))/9007199254740992 - (4872700232219253*sin(q1L))/9007199254740992))/332306998946228968225951765070086144) - (7514214926474921*cos(q4L)*((7514214926474921*cos(q3L)*((76229820211215127867025072518845*sin(q2L))/162259276829213363391578010288128 + cos(q2L)*((4872700232219253*cos(q1L))/9007199254740992 + (6283307137322267*sin(q1L))/9007199254740992) - (7514214926474921*sin(q2L)*((6283307137322267*cos(q1L))/9007199254740992 - (4872700232219253*sin(q1L))/9007199254740992))/36893488147419103232))/36893488147419103232 + sin(q3L)*((7514214926474921*cos(q2L)*((6283307137322267*cos(q1L))/9007199254740992 - (4872700232219253*sin(q1L))/9007199254740992))/36893488147419103232 - (76229820211215127867025072518845*cos(q2L))/162259276829213363391578010288128 + sin(q2L)*((4872700232219253*cos(q1L))/9007199254740992 + (6283307137322267*sin(q1L))/9007199254740992))))/36893488147419103232))/2451992865385422173373355243440494693789982595493763481600 + (3*sin(q2L)*((4872700232219253*cos(q1L))/9007199254740992 + (6283307137322267*sin(q1L))/9007199254740992))/100 + (807520961047489018778067709720399904923771262077295170375712179706208528987338271217011451790113918662491539890779991*sin(q2L)*((6283307137322267*cos(q1L))/9007199254740992 - (4872700232219253*sin(q1L))/9007199254740992))/15760802478557791684911616040057445522031895708186178667179317361698288708598884244565706501953966256322651196122726400000 + (202883803014822867*sin(q5L)*(((4503599440548691*cos(q4L))/4503599627370496 - (7514214926474921*sin(q4L))/36893488147419103232)*(cos(q3L)*((7514214926474921*cos(q2L)*((6283307137322267*cos(q1L))/9007199254740992 - (4872700232219253*sin(q1L))/9007199254740992))/36893488147419103232 - (76229820211215127867025072518845*cos(q2L))/162259276829213363391578010288128 + sin(q2L)*((4872700232219253*cos(q1L))/9007199254740992 + (6283307137322267*sin(q1L))/9007199254740992)) - (7514214926474921*sin(q3L)*((76229820211215127867025072518845*sin(q2L))/162259276829213363391578010288128 + cos(q2L)*((4872700232219253*cos(q1L))/9007199254740992 + (6283307137322267*sin(q1L))/9007199254740992) - (7514214926474921*sin(q2L)*((6283307137322267*cos(q1L))/9007199254740992 - (4872700232219253*sin(q1L))/9007199254740992))/36893488147419103232))/36893488147419103232) + ((234819211581865*cos(q4L))/1152921504606846976 + (9007199067919185*sin(q4L))/9007199254740992)*((686617165554103949950999710565799465200849541325*sin(q2L))/1461501637330902918203684832716283019655932542976 + (9007199067919185*cos(q2L)*((4872700232219253*cos(q1L))/9007199254740992 + (6283307137322267*sin(q1L))/9007199254740992))/9007199254740992 - (67682029681889335677290557259385*sin(q2L)*((6283307137322267*cos(q1L))/9007199254740992 - (4872700232219253*sin(q1L))/9007199254740992))/332306998946228968225951765070086144) - (7514214926474921*cos(q4L)*((7514214926474921*cos(q3L)*((76229820211215127867025072518845*sin(q2L))/162259276829213363391578010288128 + cos(q2L)*((4872700232219253*cos(q1L))/9007199254740992 + (6283307137322267*sin(q1L))/9007199254740992) - (7514214926474921*sin(q2L)*((6283307137322267*cos(q1L))/9007199254740992 - (4872700232219253*sin(q1L))/9007199254740992))/36893488147419103232))/36893488147419103232 + sin(q3L)*((7514214926474921*cos(q2L)*((6283307137322267*cos(q1L))/9007199254740992 - (4872700232219253*sin(q1L))/9007199254740992))/36893488147419103232 - (76229820211215127867025072518845*cos(q2L))/162259276829213363391578010288128 + sin(q2L)*((4872700232219253*cos(q1L))/9007199254740992 + (6283307137322267*sin(q1L))/9007199254740992))))/36893488147419103232))/36893488147419103232000 + (27*cos(q5L)*(((9007199067919185*cos(q4L))/9007199254740992 - (234819211581865*sin(q4L))/1152921504606846976)*((686617165554103949950999710565799465200849541325*sin(q2L))/1461501637330902918203684832716283019655932542976 + (9007199067919185*cos(q2L)*((4872700232219253*cos(q1L))/9007199254740992 + (6283307137322267*sin(q1L))/9007199254740992))/9007199254740992 - (67682029681889335677290557259385*sin(q2L)*((6283307137322267*cos(q1L))/9007199254740992 - (4872700232219253*sin(q1L))/9007199254740992))/332306998946228968225951765070086144) - ((7514214926474921*cos(q4L))/36893488147419103232 + (4503599440548691*sin(q4L))/4503599627370496)*(cos(q3L)*((7514214926474921*cos(q2L)*((6283307137322267*cos(q1L))/9007199254740992 - (4872700232219253*sin(q1L))/9007199254740992))/36893488147419103232 - (76229820211215127867025072518845*cos(q2L))/162259276829213363391578010288128 + sin(q2L)*((4872700232219253*cos(q1L))/9007199254740992 + (6283307137322267*sin(q1L))/9007199254740992)) - (7514214926474921*sin(q3L)*((76229820211215127867025072518845*sin(q2L))/162259276829213363391578010288128 + cos(q2L)*((4872700232219253*cos(q1L))/9007199254740992 + (6283307137322267*sin(q1L))/9007199254740992) - (7514214926474921*sin(q2L)*((6283307137322267*cos(q1L))/9007199254740992 - (4872700232219253*sin(q1L))/9007199254740992))/36893488147419103232))/36893488147419103232) + (7514214926474921*sin(q4L)*((7514214926474921*cos(q3L)*((76229820211215127867025072518845*sin(q2L))/162259276829213363391578010288128 + cos(q2L)*((4872700232219253*cos(q1L))/9007199254740992 + (6283307137322267*sin(q1L))/9007199254740992) - (7514214926474921*sin(q2L)*((6283307137322267*cos(q1L))/9007199254740992 - (4872700232219253*sin(q1L))/9007199254740992))/36893488147419103232))/36893488147419103232 + sin(q3L)*((7514214926474921*cos(q2L)*((6283307137322267*cos(q1L))/9007199254740992 - (4872700232219253*sin(q1L))/9007199254740992))/36893488147419103232 - (76229820211215127867025072518845*cos(q2L))/162259276829213363391578010288128 + sin(q2L)*((4872700232219253*cos(q1L))/9007199254740992 + (6283307137322267*sin(q1L))/9007199254740992))))/36893488147419103232))/1000 + (94754841554645069948206780163139*sin(q5L)*(((9007199067919185*cos(q4L))/9007199254740992 - (234819211581865*sin(q4L))/1152921504606846976)*((686617165554103949950999710565799465200849541325*sin(q2L))/1461501637330902918203684832716283019655932542976 + (9007199067919185*cos(q2L)*((4872700232219253*cos(q1L))/9007199254740992 + (6283307137322267*sin(q1L))/9007199254740992))/9007199254740992 - (67682029681889335677290557259385*sin(q2L)*((6283307137322267*cos(q1L))/9007199254740992 - (4872700232219253*sin(q1L))/9007199254740992))/332306998946228968225951765070086144) - ((7514214926474921*cos(q4L))/36893488147419103232 + (4503599440548691*sin(q4L))/4503599627370496)*(cos(q3L)*((7514214926474921*cos(q2L)*((6283307137322267*cos(q1L))/9007199254740992 - (4872700232219253*sin(q1L))/9007199254740992))/36893488147419103232 - (76229820211215127867025072518845*cos(q2L))/162259276829213363391578010288128 + sin(q2L)*((4872700232219253*cos(q1L))/9007199254740992 + (6283307137322267*sin(q1L))/9007199254740992)) - (7514214926474921*sin(q3L)*((76229820211215127867025072518845*sin(q2L))/162259276829213363391578010288128 + cos(q2L)*((4872700232219253*cos(q1L))/9007199254740992 + (6283307137322267*sin(q1L))/9007199254740992) - (7514214926474921*sin(q2L)*((6283307137322267*cos(q1L))/9007199254740992 - (4872700232219253*sin(q1L))/9007199254740992))/36893488147419103232))/36893488147419103232) + (7514214926474921*sin(q4L)*((7514214926474921*cos(q3L)*((76229820211215127867025072518845*sin(q2L))/162259276829213363391578010288128 + cos(q2L)*((4872700232219253*cos(q1L))/9007199254740992 + (6283307137322267*sin(q1L))/9007199254740992) - (7514214926474921*sin(q2L)*((6283307137322267*cos(q1L))/9007199254740992 - (4872700232219253*sin(q1L))/9007199254740992))/36893488147419103232))/36893488147419103232 + sin(q3L)*((7514214926474921*cos(q2L)*((6283307137322267*cos(q1L))/9007199254740992 - (4872700232219253*sin(q1L))/9007199254740992))/36893488147419103232 - (76229820211215127867025072518845*cos(q2L))/162259276829213363391578010288128 + sin(q2L)*((4872700232219253*cos(q1L))/9007199254740992 + (6283307137322267*sin(q1L))/9007199254740992))))/36893488147419103232))/66461399789245793645190353014017228800 - (81*((9007199067919185*cos(q4L))/9007199254740992 - (234819211581865*sin(q4L))/1152921504606846976)*((686617165554103949950999710565799465200849541325*sin(q2L))/1461501637330902918203684832716283019655932542976 + (9007199067919185*cos(q2L)*((4872700232219253*cos(q1L))/9007199254740992 + (6283307137322267*sin(q1L))/9007199254740992))/9007199254740992 - (67682029681889335677290557259385*sin(q2L)*((6283307137322267*cos(q1L))/9007199254740992 - (4872700232219253*sin(q1L))/9007199254740992))/332306998946228968225951765070086144))/2000 + (81222263116692158804177042061221826384594597321566869716687*((234819211581865*cos(q4L))/1152921504606846976 + (9007199067919185*sin(q4L))/9007199254740992)*((686617165554103949950999710565799465200849541325*sin(q2L))/1461501637330902918203684832716283019655932542976 + (9007199067919185*cos(q2L)*((4872700232219253*cos(q1L))/9007199254740992 + (6283307137322267*sin(q1L))/9007199254740992))/9007199254740992 - (67682029681889335677290557259385*sin(q2L)*((6283307137322267*cos(q1L))/9007199254740992 - (4872700232219253*sin(q1L))/9007199254740992))/332306998946228968225951765070086144))/306499108173177771671669405430061836723747824436720435200000 - (610321541873521657855151997354401418608858870661075444886782706002880706727*cos(q4L)*((7514214926474921*cos(q3L)*((76229820211215127867025072518845*sin(q2L))/162259276829213363391578010288128 + cos(q2L)*((4872700232219253*cos(q1L))/9007199254740992 + (6283307137322267*sin(q1L))/9007199254740992) - (7514214926474921*sin(q2L)*((6283307137322267*cos(q1L))/9007199254740992 - (4872700232219253*sin(q1L))/9007199254740992))/36893488147419103232))/36893488147419103232 + sin(q3L)*((7514214926474921*cos(q2L)*((6283307137322267*cos(q1L))/9007199254740992 - (4872700232219253*sin(q1L))/9007199254740992))/36893488147419103232 - (76229820211215127867025072518845*cos(q2L))/162259276829213363391578010288128 + sin(q2L)*((4872700232219253*cos(q1L))/9007199254740992 + (6283307137322267*sin(q1L))/9007199254740992))))/11307821214581659709333104004754678501295896940003961331978279688272766566400000 - (608651409044468601*sin(q4L)*((7514214926474921*cos(q3L)*((76229820211215127867025072518845*sin(q2L))/162259276829213363391578010288128 + cos(q2L)*((4872700232219253*cos(q1L))/9007199254740992 + (6283307137322267*sin(q1L))/9007199254740992) - (7514214926474921*sin(q2L)*((6283307137322267*cos(q1L))/9007199254740992 - (4872700232219253*sin(q1L))/9007199254740992))/36893488147419103232))/36893488147419103232 + sin(q3L)*((7514214926474921*cos(q2L)*((6283307137322267*cos(q1L))/9007199254740992 - (4872700232219253*sin(q1L))/9007199254740992))/36893488147419103232 - (76229820211215127867025072518845*cos(q2L))/162259276829213363391578010288128 + sin(q2L)*((4872700232219253*cos(q1L))/9007199254740992 + (6283307137322267*sin(q1L))/9007199254740992))))/73786976294838206464000 + (170695144106365826517608855445768431563113584343*cos(q5L)*((1076049180065244948668759145796765391250102872519935285209856875*sin(q2L))/55213970774324510299478046898216203619608871777363092441300193790394368 + (234819211581865*cos(q3L)*((7514214926474921*cos(q2L)*((6283307137322267*cos(q1L))/9007199254740992 - (4872700232219253*sin(q1L))/9007199254740992))/36893488147419103232 - (76229820211215127867025072518845*cos(q2L))/162259276829213363391578010288128 + sin(q2L)*((4872700232219253*cos(q1L))/9007199254740992 + (6283307137322267*sin(q1L))/9007199254740992)))/1152921504606846976 + (67682029681889335677290557259385*cos(q3L)*((76229820211215127867025072518845*sin(q2L))/162259276829213363391578010288128 + cos(q2L)*((4872700232219253*cos(q1L))/9007199254740992 + (6283307137322267*sin(q1L))/9007199254740992) - (7514214926474921*sin(q2L)*((6283307137322267*cos(q1L))/9007199254740992 - (4872700232219253*sin(q1L))/9007199254740992))/36893488147419103232))/332306998946228968225951765070086144 + (9007199067919185*sin(q3L)*((7514214926474921*cos(q2L)*((6283307137322267*cos(q1L))/9007199254740992 - (4872700232219253*sin(q1L))/9007199254740992))/36893488147419103232 - (76229820211215127867025072518845*cos(q2L))/162259276829213363391578010288128 + sin(q2L)*((4872700232219253*cos(q1L))/9007199254740992 + (6283307137322267*sin(q1L))/9007199254740992)))/9007199254740992 - (1764482024691522628700660907665*sin(q3L)*((76229820211215127867025072518845*sin(q2L))/162259276829213363391578010288128 + cos(q2L)*((4872700232219253*cos(q1L))/9007199254740992 + (6283307137322267*sin(q1L))/9007199254740992) - (7514214926474921*sin(q2L)*((6283307137322267*cos(q1L))/9007199254740992 - (4872700232219253*sin(q1L))/9007199254740992))/36893488147419103232))/42535295865117307932921825928971026432 + (14115856197532180673579726082375*cos(q2L)*((4872700232219253*cos(q1L))/9007199254740992 + (6283307137322267*sin(q1L))/9007199254740992))/340282366920938463463374607431768211456 - (106069577339469832923929692356850887620017617375*sin(q2L)*((6283307137322267*cos(q1L))/9007199254740992 - (4872700232219253*sin(q1L))/9007199254740992))/12554203470773361527671578846415332832204710888928069025792))/119726214130147567059245861496117904970213993920593920 - (48638874966763599*sin(q5L)*((1076049180065244948668759145796765391250102872519935285209856875*sin(q2L))/55213970774324510299478046898216203619608871777363092441300193790394368 + (234819211581865*cos(q3L)*((7514214926474921*cos(q2L)*((6283307137322267*cos(q1L))/9007199254740992 - (4872700232219253*sin(q1L))/9007199254740992))/36893488147419103232 - (76229820211215127867025072518845*cos(q2L))/162259276829213363391578010288128 + sin(q2L)*((4872700232219253*cos(q1L))/9007199254740992 + (6283307137322267*sin(q1L))/9007199254740992)))/1152921504606846976 + (67682029681889335677290557259385*cos(q3L)*((76229820211215127867025072518845*sin(q2L))/162259276829213363391578010288128 + cos(q2L)*((4872700232219253*cos(q1L))/9007199254740992 + (6283307137322267*sin(q1L))/9007199254740992) - (7514214926474921*sin(q2L)*((6283307137322267*cos(q1L))/9007199254740992 - (4872700232219253*sin(q1L))/9007199254740992))/36893488147419103232))/332306998946228968225951765070086144 + (9007199067919185*sin(q3L)*((7514214926474921*cos(q2L)*((6283307137322267*cos(q1L))/9007199254740992 - (4872700232219253*sin(q1L))/9007199254740992))/36893488147419103232 - (76229820211215127867025072518845*cos(q2L))/162259276829213363391578010288128 + sin(q2L)*((4872700232219253*cos(q1L))/9007199254740992 + (6283307137322267*sin(q1L))/9007199254740992)))/9007199254740992 - (1764482024691522628700660907665*sin(q3L)*((76229820211215127867025072518845*sin(q2L))/162259276829213363391578010288128 + cos(q2L)*((4872700232219253*cos(q1L))/9007199254740992 + (6283307137322267*sin(q1L))/9007199254740992) - (7514214926474921*sin(q2L)*((6283307137322267*cos(q1L))/9007199254740992 - (4872700232219253*sin(q1L))/9007199254740992))/36893488147419103232))/42535295865117307932921825928971026432 + (14115856197532180673579726082375*cos(q2L)*((4872700232219253*cos(q1L))/9007199254740992 + (6283307137322267*sin(q1L))/9007199254740992))/340282366920938463463374607431768211456 - (106069577339469832923929692356850887620017617375*sin(q2L)*((6283307137322267*cos(q1L))/9007199254740992 - (4872700232219253*sin(q1L))/9007199254740992))/12554203470773361527671578846415332832204710888928069025792))/1801439850948198400 - (2436553109258773196144549622003023*cos(q6L)*(sin(q5L)*(((9007199067919185*cos(q4L))/9007199254740992 - (234819211581865*sin(q4L))/1152921504606846976)*((686617165554103949950999710565799465200849541325*sin(q2L))/1461501637330902918203684832716283019655932542976 + (9007199067919185*cos(q2L)*((4872700232219253*cos(q1L))/9007199254740992 + (6283307137322267*sin(q1L))/9007199254740992))/9007199254740992 - (67682029681889335677290557259385*sin(q2L)*((6283307137322267*cos(q1L))/9007199254740992 - (4872700232219253*sin(q1L))/9007199254740992))/332306998946228968225951765070086144) - ((7514214926474921*cos(q4L))/36893488147419103232 + (4503599440548691*sin(q4L))/4503599627370496)*(cos(q3L)*((7514214926474921*cos(q2L)*((6283307137322267*cos(q1L))/9007199254740992 - (4872700232219253*sin(q1L))/9007199254740992))/36893488147419103232 - (76229820211215127867025072518845*cos(q2L))/162259276829213363391578010288128 + sin(q2L)*((4872700232219253*cos(q1L))/9007199254740992 + (6283307137322267*sin(q1L))/9007199254740992)) - (7514214926474921*sin(q3L)*((76229820211215127867025072518845*sin(q2L))/162259276829213363391578010288128 + cos(q2L)*((4872700232219253*cos(q1L))/9007199254740992 + (6283307137322267*sin(q1L))/9007199254740992) - (7514214926474921*sin(q2L)*((6283307137322267*cos(q1L))/9007199254740992 - (4872700232219253*sin(q1L))/9007199254740992))/36893488147419103232))/36893488147419103232) + (7514214926474921*sin(q4L)*((7514214926474921*cos(q3L)*((76229820211215127867025072518845*sin(q2L))/162259276829213363391578010288128 + cos(q2L)*((4872700232219253*cos(q1L))/9007199254740992 + (6283307137322267*sin(q1L))/9007199254740992) - (7514214926474921*sin(q2L)*((6283307137322267*cos(q1L))/9007199254740992 - (4872700232219253*sin(q1L))/9007199254740992))/36893488147419103232))/36893488147419103232 + sin(q3L)*((7514214926474921*cos(q2L)*((6283307137322267*cos(q1L))/9007199254740992 - (4872700232219253*sin(q1L))/9007199254740992))/36893488147419103232 - (76229820211215127867025072518845*cos(q2L))/162259276829213363391578010288128 + sin(q2L)*((4872700232219253*cos(q1L))/9007199254740992 + (6283307137322267*sin(q1L))/9007199254740992))))/36893488147419103232) - (7514214926474921*cos(q5L)*(((4503599440548691*cos(q4L))/4503599627370496 - (7514214926474921*sin(q4L))/36893488147419103232)*(cos(q3L)*((7514214926474921*cos(q2L)*((6283307137322267*cos(q1L))/9007199254740992 - (4872700232219253*sin(q1L))/9007199254740992))/36893488147419103232 - (76229820211215127867025072518845*cos(q2L))/162259276829213363391578010288128 + sin(q2L)*((4872700232219253*cos(q1L))/9007199254740992 + (6283307137322267*sin(q1L))/9007199254740992)) - (7514214926474921*sin(q3L)*((76229820211215127867025072518845*sin(q2L))/162259276829213363391578010288128 + cos(q2L)*((4872700232219253*cos(q1L))/9007199254740992 + (6283307137322267*sin(q1L))/9007199254740992) - (7514214926474921*sin(q2L)*((6283307137322267*cos(q1L))/9007199254740992 - (4872700232219253*sin(q1L))/9007199254740992))/36893488147419103232))/36893488147419103232) + ((234819211581865*cos(q4L))/1152921504606846976 + (9007199067919185*sin(q4L))/9007199254740992)*((686617165554103949950999710565799465200849541325*sin(q2L))/1461501637330902918203684832716283019655932542976 + (9007199067919185*cos(q2L)*((4872700232219253*cos(q1L))/9007199254740992 + (6283307137322267*sin(q1L))/9007199254740992))/9007199254740992 - (67682029681889335677290557259385*sin(q2L)*((6283307137322267*cos(q1L))/9007199254740992 - (4872700232219253*sin(q1L))/9007199254740992))/332306998946228968225951765070086144) - (7514214926474921*cos(q4L)*((7514214926474921*cos(q3L)*((76229820211215127867025072518845*sin(q2L))/162259276829213363391578010288128 + cos(q2L)*((4872700232219253*cos(q1L))/9007199254740992 + (6283307137322267*sin(q1L))/9007199254740992) - (7514214926474921*sin(q2L)*((6283307137322267*cos(q1L))/9007199254740992 - (4872700232219253*sin(q1L))/9007199254740992))/36893488147419103232))/36893488147419103232 + sin(q3L)*((7514214926474921*cos(q2L)*((6283307137322267*cos(q1L))/9007199254740992 - (4872700232219253*sin(q1L))/9007199254740992))/36893488147419103232 - (76229820211215127867025072518845*cos(q2L))/162259276829213363391578010288128 + sin(q2L)*((4872700232219253*cos(q1L))/9007199254740992 + (6283307137322267*sin(q1L))/9007199254740992))))/36893488147419103232))/36893488147419103232 + (9007199067919185*cos(q5L)*((1076049180065244948668759145796765391250102872519935285209856875*sin(q2L))/55213970774324510299478046898216203619608871777363092441300193790394368 + (234819211581865*cos(q3L)*((7514214926474921*cos(q2L)*((6283307137322267*cos(q1L))/9007199254740992 - (4872700232219253*sin(q1L))/9007199254740992))/36893488147419103232 - (76229820211215127867025072518845*cos(q2L))/162259276829213363391578010288128 + sin(q2L)*((4872700232219253*cos(q1L))/9007199254740992 + (6283307137322267*sin(q1L))/9007199254740992)))/1152921504606846976 + (67682029681889335677290557259385*cos(q3L)*((76229820211215127867025072518845*sin(q2L))/162259276829213363391578010288128 + cos(q2L)*((4872700232219253*cos(q1L))/9007199254740992 + (6283307137322267*sin(q1L))/9007199254740992) - (7514214926474921*sin(q2L)*((6283307137322267*cos(q1L))/9007199254740992 - (4872700232219253*sin(q1L))/9007199254740992))/36893488147419103232))/332306998946228968225951765070086144 + (9007199067919185*sin(q3L)*((7514214926474921*cos(q2L)*((6283307137322267*cos(q1L))/9007199254740992 - (4872700232219253*sin(q1L))/9007199254740992))/36893488147419103232 - (76229820211215127867025072518845*cos(q2L))/162259276829213363391578010288128 + sin(q2L)*((4872700232219253*cos(q1L))/9007199254740992 + (6283307137322267*sin(q1L))/9007199254740992)))/9007199254740992 - (1764482024691522628700660907665*sin(q3L)*((76229820211215127867025072518845*sin(q2L))/162259276829213363391578010288128 + cos(q2L)*((4872700232219253*cos(q1L))/9007199254740992 + (6283307137322267*sin(q1L))/9007199254740992) - (7514214926474921*sin(q2L)*((6283307137322267*cos(q1L))/9007199254740992 - (4872700232219253*sin(q1L))/9007199254740992))/36893488147419103232))/42535295865117307932921825928971026432 + (14115856197532180673579726082375*cos(q2L)*((4872700232219253*cos(q1L))/9007199254740992 + (6283307137322267*sin(q1L))/9007199254740992))/340282366920938463463374607431768211456 - (106069577339469832923929692356850887620017617375*sin(q2L)*((6283307137322267*cos(q1L))/9007199254740992 - (4872700232219253*sin(q1L))/9007199254740992))/12554203470773361527671578846415332832204710888928069025792))/9007199254740992))/332306998946228968225951765070086144000 - (27*cos(q6L)*((7514214926474921*sin(q5L)*(((4503599440548691*cos(q4L))/4503599627370496 - (7514214926474921*sin(q4L))/36893488147419103232)*(cos(q3L)*((7514214926474921*cos(q2L)*((6283307137322267*cos(q1L))/9007199254740992 - (4872700232219253*sin(q1L))/9007199254740992))/36893488147419103232 - (76229820211215127867025072518845*cos(q2L))/162259276829213363391578010288128 + sin(q2L)*((4872700232219253*cos(q1L))/9007199254740992 + (6283307137322267*sin(q1L))/9007199254740992)) - (7514214926474921*sin(q3L)*((76229820211215127867025072518845*sin(q2L))/162259276829213363391578010288128 + cos(q2L)*((4872700232219253*cos(q1L))/9007199254740992 + (6283307137322267*sin(q1L))/9007199254740992) - (7514214926474921*sin(q2L)*((6283307137322267*cos(q1L))/9007199254740992 - (4872700232219253*sin(q1L))/9007199254740992))/36893488147419103232))/36893488147419103232) + ((234819211581865*cos(q4L))/1152921504606846976 + (9007199067919185*sin(q4L))/9007199254740992)*((686617165554103949950999710565799465200849541325*sin(q2L))/1461501637330902918203684832716283019655932542976 + (9007199067919185*cos(q2L)*((4872700232219253*cos(q1L))/9007199254740992 + (6283307137322267*sin(q1L))/9007199254740992))/9007199254740992 - (67682029681889335677290557259385*sin(q2L)*((6283307137322267*cos(q1L))/9007199254740992 - (4872700232219253*sin(q1L))/9007199254740992))/332306998946228968225951765070086144) - (7514214926474921*cos(q4L)*((7514214926474921*cos(q3L)*((76229820211215127867025072518845*sin(q2L))/162259276829213363391578010288128 + cos(q2L)*((4872700232219253*cos(q1L))/9007199254740992 + (6283307137322267*sin(q1L))/9007199254740992) - (7514214926474921*sin(q2L)*((6283307137322267*cos(q1L))/9007199254740992 - (4872700232219253*sin(q1L))/9007199254740992))/36893488147419103232))/36893488147419103232 + sin(q3L)*((7514214926474921*cos(q2L)*((6283307137322267*cos(q1L))/9007199254740992 - (4872700232219253*sin(q1L))/9007199254740992))/36893488147419103232 - (76229820211215127867025072518845*cos(q2L))/162259276829213363391578010288128 + sin(q2L)*((4872700232219253*cos(q1L))/9007199254740992 + (6283307137322267*sin(q1L))/9007199254740992))))/36893488147419103232))/36893488147419103232 + cos(q5L)*(((9007199067919185*cos(q4L))/9007199254740992 - (234819211581865*sin(q4L))/1152921504606846976)*((686617165554103949950999710565799465200849541325*sin(q2L))/1461501637330902918203684832716283019655932542976 + (9007199067919185*cos(q2L)*((4872700232219253*cos(q1L))/9007199254740992 + (6283307137322267*sin(q1L))/9007199254740992))/9007199254740992 - (67682029681889335677290557259385*sin(q2L)*((6283307137322267*cos(q1L))/9007199254740992 - (4872700232219253*sin(q1L))/9007199254740992))/332306998946228968225951765070086144) - ((7514214926474921*cos(q4L))/36893488147419103232 + (4503599440548691*sin(q4L))/4503599627370496)*(cos(q3L)*((7514214926474921*cos(q2L)*((6283307137322267*cos(q1L))/9007199254740992 - (4872700232219253*sin(q1L))/9007199254740992))/36893488147419103232 - (76229820211215127867025072518845*cos(q2L))/162259276829213363391578010288128 + sin(q2L)*((4872700232219253*cos(q1L))/9007199254740992 + (6283307137322267*sin(q1L))/9007199254740992)) - (7514214926474921*sin(q3L)*((76229820211215127867025072518845*sin(q2L))/162259276829213363391578010288128 + cos(q2L)*((4872700232219253*cos(q1L))/9007199254740992 + (6283307137322267*sin(q1L))/9007199254740992) - (7514214926474921*sin(q2L)*((6283307137322267*cos(q1L))/9007199254740992 - (4872700232219253*sin(q1L))/9007199254740992))/36893488147419103232))/36893488147419103232) + (7514214926474921*sin(q4L)*((7514214926474921*cos(q3L)*((76229820211215127867025072518845*sin(q2L))/162259276829213363391578010288128 + cos(q2L)*((4872700232219253*cos(q1L))/9007199254740992 + (6283307137322267*sin(q1L))/9007199254740992) - (7514214926474921*sin(q2L)*((6283307137322267*cos(q1L))/9007199254740992 - (4872700232219253*sin(q1L))/9007199254740992))/36893488147419103232))/36893488147419103232 + sin(q3L)*((7514214926474921*cos(q2L)*((6283307137322267*cos(q1L))/9007199254740992 - (4872700232219253*sin(q1L))/9007199254740992))/36893488147419103232 - (76229820211215127867025072518845*cos(q2L))/162259276829213363391578010288128 + sin(q2L)*((4872700232219253*cos(q1L))/9007199254740992 + (6283307137322267*sin(q1L))/9007199254740992))))/36893488147419103232) - (9007199067919185*sin(q5L)*((1076049180065244948668759145796765391250102872519935285209856875*sin(q2L))/55213970774324510299478046898216203619608871777363092441300193790394368 + (234819211581865*cos(q3L)*((7514214926474921*cos(q2L)*((6283307137322267*cos(q1L))/9007199254740992 - (4872700232219253*sin(q1L))/9007199254740992))/36893488147419103232 - (76229820211215127867025072518845*cos(q2L))/162259276829213363391578010288128 + sin(q2L)*((4872700232219253*cos(q1L))/9007199254740992 + (6283307137322267*sin(q1L))/9007199254740992)))/1152921504606846976 + (67682029681889335677290557259385*cos(q3L)*((76229820211215127867025072518845*sin(q2L))/162259276829213363391578010288128 + cos(q2L)*((4872700232219253*cos(q1L))/9007199254740992 + (6283307137322267*sin(q1L))/9007199254740992) - (7514214926474921*sin(q2L)*((6283307137322267*cos(q1L))/9007199254740992 - (4872700232219253*sin(q1L))/9007199254740992))/36893488147419103232))/332306998946228968225951765070086144 + (9007199067919185*sin(q3L)*((7514214926474921*cos(q2L)*((6283307137322267*cos(q1L))/9007199254740992 - (4872700232219253*sin(q1L))/9007199254740992))/36893488147419103232 - (76229820211215127867025072518845*cos(q2L))/162259276829213363391578010288128 + sin(q2L)*((4872700232219253*cos(q1L))/9007199254740992 + (6283307137322267*sin(q1L))/9007199254740992)))/9007199254740992 - (1764482024691522628700660907665*sin(q3L)*((76229820211215127867025072518845*sin(q2L))/162259276829213363391578010288128 + cos(q2L)*((4872700232219253*cos(q1L))/9007199254740992 + (6283307137322267*sin(q1L))/9007199254740992) - (7514214926474921*sin(q2L)*((6283307137322267*cos(q1L))/9007199254740992 - (4872700232219253*sin(q1L))/9007199254740992))/36893488147419103232))/42535295865117307932921825928971026432 + (14115856197532180673579726082375*cos(q2L)*((4872700232219253*cos(q1L))/9007199254740992 + (6283307137322267*sin(q1L))/9007199254740992))/340282366920938463463374607431768211456 - (106069577339469832923929692356850887620017617375*sin(q2L)*((6283307137322267*cos(q1L))/9007199254740992 - (4872700232219253*sin(q1L))/9007199254740992))/12554203470773361527671578846415332832204710888928069025792))/9007199254740992))/1000 - (202883803014822867*sin(q6L)*(sin(q5L)*(((9007199067919185*cos(q4L))/9007199254740992 - (234819211581865*sin(q4L))/1152921504606846976)*((686617165554103949950999710565799465200849541325*sin(q2L))/1461501637330902918203684832716283019655932542976 + (9007199067919185*cos(q2L)*((4872700232219253*cos(q1L))/9007199254740992 + (6283307137322267*sin(q1L))/9007199254740992))/9007199254740992 - (67682029681889335677290557259385*sin(q2L)*((6283307137322267*cos(q1L))/9007199254740992 - (4872700232219253*sin(q1L))/9007199254740992))/332306998946228968225951765070086144) - ((7514214926474921*cos(q4L))/36893488147419103232 + (4503599440548691*sin(q4L))/4503599627370496)*(cos(q3L)*((7514214926474921*cos(q2L)*((6283307137322267*cos(q1L))/9007199254740992 - (4872700232219253*sin(q1L))/9007199254740992))/36893488147419103232 - (76229820211215127867025072518845*cos(q2L))/162259276829213363391578010288128 + sin(q2L)*((4872700232219253*cos(q1L))/9007199254740992 + (6283307137322267*sin(q1L))/9007199254740992)) - (7514214926474921*sin(q3L)*((76229820211215127867025072518845*sin(q2L))/162259276829213363391578010288128 + cos(q2L)*((4872700232219253*cos(q1L))/9007199254740992 + (6283307137322267*sin(q1L))/9007199254740992) - (7514214926474921*sin(q2L)*((6283307137322267*cos(q1L))/9007199254740992 - (4872700232219253*sin(q1L))/9007199254740992))/36893488147419103232))/36893488147419103232) + (7514214926474921*sin(q4L)*((7514214926474921*cos(q3L)*((76229820211215127867025072518845*sin(q2L))/162259276829213363391578010288128 + cos(q2L)*((4872700232219253*cos(q1L))/9007199254740992 + (6283307137322267*sin(q1L))/9007199254740992) - (7514214926474921*sin(q2L)*((6283307137322267*cos(q1L))/9007199254740992 - (4872700232219253*sin(q1L))/9007199254740992))/36893488147419103232))/36893488147419103232 + sin(q3L)*((7514214926474921*cos(q2L)*((6283307137322267*cos(q1L))/9007199254740992 - (4872700232219253*sin(q1L))/9007199254740992))/36893488147419103232 - (76229820211215127867025072518845*cos(q2L))/162259276829213363391578010288128 + sin(q2L)*((4872700232219253*cos(q1L))/9007199254740992 + (6283307137322267*sin(q1L))/9007199254740992))))/36893488147419103232) - (7514214926474921*cos(q5L)*(((4503599440548691*cos(q4L))/4503599627370496 - (7514214926474921*sin(q4L))/36893488147419103232)*(cos(q3L)*((7514214926474921*cos(q2L)*((6283307137322267*cos(q1L))/9007199254740992 - (4872700232219253*sin(q1L))/9007199254740992))/36893488147419103232 - (76229820211215127867025072518845*cos(q2L))/162259276829213363391578010288128 + sin(q2L)*((4872700232219253*cos(q1L))/9007199254740992 + (6283307137322267*sin(q1L))/9007199254740992)) - (7514214926474921*sin(q3L)*((76229820211215127867025072518845*sin(q2L))/162259276829213363391578010288128 + cos(q2L)*((4872700232219253*cos(q1L))/9007199254740992 + (6283307137322267*sin(q1L))/9007199254740992) - (7514214926474921*sin(q2L)*((6283307137322267*cos(q1L))/9007199254740992 - (4872700232219253*sin(q1L))/9007199254740992))/36893488147419103232))/36893488147419103232) + ((234819211581865*cos(q4L))/1152921504606846976 + (9007199067919185*sin(q4L))/9007199254740992)*((686617165554103949950999710565799465200849541325*sin(q2L))/1461501637330902918203684832716283019655932542976 + (9007199067919185*cos(q2L)*((4872700232219253*cos(q1L))/9007199254740992 + (6283307137322267*sin(q1L))/9007199254740992))/9007199254740992 - (67682029681889335677290557259385*sin(q2L)*((6283307137322267*cos(q1L))/9007199254740992 - (4872700232219253*sin(q1L))/9007199254740992))/332306998946228968225951765070086144) - (7514214926474921*cos(q4L)*((7514214926474921*cos(q3L)*((76229820211215127867025072518845*sin(q2L))/162259276829213363391578010288128 + cos(q2L)*((4872700232219253*cos(q1L))/9007199254740992 + (6283307137322267*sin(q1L))/9007199254740992) - (7514214926474921*sin(q2L)*((6283307137322267*cos(q1L))/9007199254740992 - (4872700232219253*sin(q1L))/9007199254740992))/36893488147419103232))/36893488147419103232 + sin(q3L)*((7514214926474921*cos(q2L)*((6283307137322267*cos(q1L))/9007199254740992 - (4872700232219253*sin(q1L))/9007199254740992))/36893488147419103232 - (76229820211215127867025072518845*cos(q2L))/162259276829213363391578010288128 + sin(q2L)*((4872700232219253*cos(q1L))/9007199254740992 + (6283307137322267*sin(q1L))/9007199254740992))))/36893488147419103232))/36893488147419103232 + (9007199067919185*cos(q5L)*((1076049180065244948668759145796765391250102872519935285209856875*sin(q2L))/55213970774324510299478046898216203619608871777363092441300193790394368 + (234819211581865*cos(q3L)*((7514214926474921*cos(q2L)*((6283307137322267*cos(q1L))/9007199254740992 - (4872700232219253*sin(q1L))/9007199254740992))/36893488147419103232 - (76229820211215127867025072518845*cos(q2L))/162259276829213363391578010288128 + sin(q2L)*((4872700232219253*cos(q1L))/9007199254740992 + (6283307137322267*sin(q1L))/9007199254740992)))/1152921504606846976 + (67682029681889335677290557259385*cos(q3L)*((76229820211215127867025072518845*sin(q2L))/162259276829213363391578010288128 + cos(q2L)*((4872700232219253*cos(q1L))/9007199254740992 + (6283307137322267*sin(q1L))/9007199254740992) - (7514214926474921*sin(q2L)*((6283307137322267*cos(q1L))/9007199254740992 - (4872700232219253*sin(q1L))/9007199254740992))/36893488147419103232))/332306998946228968225951765070086144 + (9007199067919185*sin(q3L)*((7514214926474921*cos(q2L)*((6283307137322267*cos(q1L))/9007199254740992 - (4872700232219253*sin(q1L))/9007199254740992))/36893488147419103232 - (76229820211215127867025072518845*cos(q2L))/162259276829213363391578010288128 + sin(q2L)*((4872700232219253*cos(q1L))/9007199254740992 + (6283307137322267*sin(q1L))/9007199254740992)))/9007199254740992 - (1764482024691522628700660907665*sin(q3L)*((76229820211215127867025072518845*sin(q2L))/162259276829213363391578010288128 + cos(q2L)*((4872700232219253*cos(q1L))/9007199254740992 + (6283307137322267*sin(q1L))/9007199254740992) - (7514214926474921*sin(q2L)*((6283307137322267*cos(q1L))/9007199254740992 - (4872700232219253*sin(q1L))/9007199254740992))/36893488147419103232))/42535295865117307932921825928971026432 + (14115856197532180673579726082375*cos(q2L)*((4872700232219253*cos(q1L))/9007199254740992 + (6283307137322267*sin(q1L))/9007199254740992))/340282366920938463463374607431768211456 - (106069577339469832923929692356850887620017617375*sin(q2L)*((6283307137322267*cos(q1L))/9007199254740992 - (4872700232219253*sin(q1L))/9007199254740992))/12554203470773361527671578846415332832204710888928069025792))/9007199254740992))/36893488147419103232000, (60617164743372705924380750591060836759586313939367162716784907429017787816377231*sin(q3L)*((76229820211215127867025072518845*sin(q2L))/162259276829213363391578010288128 + cos(q2L)*((4872700232219253*cos(q1L))/9007199254740992 + (6283307137322267*sin(q1L))/9007199254740992) - (7514214926474921*sin(q2L)*((6283307137322267*cos(q1L))/9007199254740992 - (4872700232219253*sin(q1L))/9007199254740992))/36893488147419103232))/1447401115466452442794637312608598848165874808320507050493219800098914120499200000 - (83301539375654672537075965313343183841442266989297270401707771044036658496661398777306991*sin(q3L)*((56594998190739085871744456992395*cos(q1L))/81129638414606681695789005144064 - (43889380989894851923989405068805*sin(q1L))/81129638414606681695789005144064 + 63594381400292563045725890951477/664613997892457936451903530140172288))/4074071952668972172536891376818756322102936787331872501272280898708762599526673412366794752000 - (81222263116692158804177042061221826384594597321566869716687*((4503599440548691*cos(q4L))/4503599627370496 - (7514214926474921*sin(q4L))/36893488147419103232)*((9007199067919185*cos(q3L)*((56594998190739085871744456992395*cos(q1L))/81129638414606681695789005144064 - (43889380989894851923989405068805*sin(q1L))/81129638414606681695789005144064 + 63594381400292563045725890951477/664613997892457936451903530140172288))/9007199254740992 + (7514214926474921*cos(q3L)*((7514214926474921*cos(q2L)*((6283307137322267*cos(q1L))/9007199254740992 - (4872700232219253*sin(q1L))/9007199254740992))/36893488147419103232 - (76229820211215127867025072518845*cos(q2L))/162259276829213363391578010288128 + sin(q2L)*((4872700232219253*cos(q1L))/9007199254740992 + (6283307137322267*sin(q1L))/9007199254740992)))/36893488147419103232 - sin(q3L)*((76229820211215127867025072518845*sin(q2L))/162259276829213363391578010288128 + cos(q2L)*((4872700232219253*cos(q1L))/9007199254740992 + (6283307137322267*sin(q1L))/9007199254740992) - (7514214926474921*sin(q2L)*((6283307137322267*cos(q1L))/9007199254740992 - (4872700232219253*sin(q1L))/9007199254740992))/36893488147419103232)))/306499108173177771671669405430061836723747824436720435200000 - (81*((7514214926474921*cos(q4L))/36893488147419103232 + (4503599440548691*sin(q4L))/4503599627370496)*((9007199067919185*cos(q3L)*((56594998190739085871744456992395*cos(q1L))/81129638414606681695789005144064 - (43889380989894851923989405068805*sin(q1L))/81129638414606681695789005144064 + 63594381400292563045725890951477/664613997892457936451903530140172288))/9007199254740992 + (7514214926474921*cos(q3L)*((7514214926474921*cos(q2L)*((6283307137322267*cos(q1L))/9007199254740992 - (4872700232219253*sin(q1L))/9007199254740992))/36893488147419103232 - (76229820211215127867025072518845*cos(q2L))/162259276829213363391578010288128 + sin(q2L)*((4872700232219253*cos(q1L))/9007199254740992 + (6283307137322267*sin(q1L))/9007199254740992)))/36893488147419103232 - sin(q3L)*((76229820211215127867025072518845*sin(q2L))/162259276829213363391578010288128 + cos(q2L)*((4872700232219253*cos(q1L))/9007199254740992 + (6283307137322267*sin(q1L))/9007199254740992) - (7514214926474921*sin(q2L)*((6283307137322267*cos(q1L))/9007199254740992 - (4872700232219253*sin(q1L))/9007199254740992))/36893488147419103232)))/2000 - (455490404115240510935077772268745492204390157443214084883134054419271951750419293234291596923751*cos(q3L)*((7514214926474921*cos(q2L)*((6283307137322267*cos(q1L))/9007199254740992 - (4872700232219253*sin(q1L))/9007199254740992))/36893488147419103232 - (76229820211215127867025072518845*cos(q2L))/162259276829213363391578010288128 + sin(q2L)*((4872700232219253*cos(q1L))/9007199254740992 + (6283307137322267*sin(q1L))/9007199254740992)))/53399675898022752059875542654238802865067613058916319248676040195555493144516013750574052173414400000 - (46241644459901303158631016767207157814229090534989303509431886332469146043*cos(q3L)*((76229820211215127867025072518845*sin(q2L))/162259276829213363391578010288128 + cos(q2L)*((4872700232219253*cos(q1L))/9007199254740992 + (6283307137322267*sin(q1L))/9007199254740992) - (7514214926474921*sin(q2L)*((6283307137322267*cos(q1L))/9007199254740992 - (4872700232219253*sin(q1L))/9007199254740992))/36893488147419103232))/2261564242916331941866620800950935700259179388000792266395655937654553313280000 - (347469655025336708709976918716104493695816557877713443586884917071777956519687017125887603*sin(q3L)*((7514214926474921*cos(q2L)*((6283307137322267*cos(q1L))/9007199254740992 - (4872700232219253*sin(q1L))/9007199254740992))/36893488147419103232 - (76229820211215127867025072518845*cos(q2L))/162259276829213363391578010288128 + sin(q2L)*((4872700232219253*cos(q1L))/9007199254740992 + (6283307137322267*sin(q1L))/9007199254740992)))/83436993590660550093555535397248129476668145404556748826056312805555458038306271485271956520960000 - (2436553109258773196144549622003023*cos(q6L)*((7514214926474921*cos(q5L)*(((4503599440548691*cos(q4L))/4503599627370496 - (7514214926474921*sin(q4L))/36893488147419103232)*((9007199067919185*cos(q3L)*((56594998190739085871744456992395*cos(q1L))/81129638414606681695789005144064 - (43889380989894851923989405068805*sin(q1L))/81129638414606681695789005144064 + 63594381400292563045725890951477/664613997892457936451903530140172288))/9007199254740992 + (7514214926474921*cos(q3L)*((7514214926474921*cos(q2L)*((6283307137322267*cos(q1L))/9007199254740992 - (4872700232219253*sin(q1L))/9007199254740992))/36893488147419103232 - (76229820211215127867025072518845*cos(q2L))/162259276829213363391578010288128 + sin(q2L)*((4872700232219253*cos(q1L))/9007199254740992 + (6283307137322267*sin(q1L))/9007199254740992)))/36893488147419103232 - sin(q3L)*((76229820211215127867025072518845*sin(q2L))/162259276829213363391578010288128 + cos(q2L)*((4872700232219253*cos(q1L))/9007199254740992 + (6283307137322267*sin(q1L))/9007199254740992) - (7514214926474921*sin(q2L)*((6283307137322267*cos(q1L))/9007199254740992 - (4872700232219253*sin(q1L))/9007199254740992))/36893488147419103232)) - (7514214926474921*cos(q4L)*((9007199067919185*sin(q3L)*((56594998190739085871744456992395*cos(q1L))/81129638414606681695789005144064 - (43889380989894851923989405068805*sin(q1L))/81129638414606681695789005144064 + 63594381400292563045725890951477/664613997892457936451903530140172288))/9007199254740992 + cos(q3L)*((76229820211215127867025072518845*sin(q2L))/162259276829213363391578010288128 + cos(q2L)*((4872700232219253*cos(q1L))/9007199254740992 + (6283307137322267*sin(q1L))/9007199254740992) - (7514214926474921*sin(q2L)*((6283307137322267*cos(q1L))/9007199254740992 - (4872700232219253*sin(q1L))/9007199254740992))/36893488147419103232) + (7514214926474921*sin(q3L)*((7514214926474921*cos(q2L)*((6283307137322267*cos(q1L))/9007199254740992 - (4872700232219253*sin(q1L))/9007199254740992))/36893488147419103232 - (76229820211215127867025072518845*cos(q2L))/162259276829213363391578010288128 + sin(q2L)*((4872700232219253*cos(q1L))/9007199254740992 + (6283307137322267*sin(q1L))/9007199254740992)))/36893488147419103232))/36893488147419103232))/36893488147419103232 - (9007199067919185*cos(q5L)*((2115063383689692319117831580025*cos(q3L)*((56594998190739085871744456992395*cos(q1L))/81129638414606681695789005144064 - (43889380989894851923989405068805*sin(q1L))/81129638414606681695789005144064 + 63594381400292563045725890951477/664613997892457936451903530140172288))/10384593717069655257060992658440192 + (81129635049124235038645691064225*sin(q3L)*((56594998190739085871744456992395*cos(q1L))/81129638414606681695789005144064 - (43889380989894851923989405068805*sin(q1L))/81129638414606681695789005144064 + 63594381400292563045725890951477/664613997892457936451903530140172288))/81129638414606681695789005144064 + (1764482024691522628700660907665*cos(q3L)*((7514214926474921*cos(q2L)*((6283307137322267*cos(q1L))/9007199254740992 - (4872700232219253*sin(q1L))/9007199254740992))/36893488147419103232 - (76229820211215127867025072518845*cos(q2L))/162259276829213363391578010288128 + sin(q2L)*((4872700232219253*cos(q1L))/9007199254740992 + (6283307137322267*sin(q1L))/9007199254740992)))/42535295865117307932921825928971026432 + (9007199067919185*cos(q3L)*((76229820211215127867025072518845*sin(q2L))/162259276829213363391578010288128 + cos(q2L)*((4872700232219253*cos(q1L))/9007199254740992 + (6283307137322267*sin(q1L))/9007199254740992) - (7514214926474921*sin(q2L)*((6283307137322267*cos(q1L))/9007199254740992 - (4872700232219253*sin(q1L))/9007199254740992))/36893488147419103232))/9007199254740992 + (67682029681889335677290557259385*sin(q3L)*((7514214926474921*cos(q2L)*((6283307137322267*cos(q1L))/9007199254740992 - (4872700232219253*sin(q1L))/9007199254740992))/36893488147419103232 - (76229820211215127867025072518845*cos(q2L))/162259276829213363391578010288128 + sin(q2L)*((4872700232219253*cos(q1L))/9007199254740992 + (6283307137322267*sin(q1L))/9007199254740992)))/332306998946228968225951765070086144 - (234819211581865*sin(q3L)*((76229820211215127867025072518845*sin(q2L))/162259276829213363391578010288128 + cos(q2L)*((4872700232219253*cos(q1L))/9007199254740992 + (6283307137322267*sin(q1L))/9007199254740992) - (7514214926474921*sin(q2L)*((6283307137322267*cos(q1L))/9007199254740992 - (4872700232219253*sin(q1L))/9007199254740992))/36893488147419103232))/1152921504606846976))/9007199254740992 + sin(q5L)*(((7514214926474921*cos(q4L))/36893488147419103232 + (4503599440548691*sin(q4L))/4503599627370496)*((9007199067919185*cos(q3L)*((56594998190739085871744456992395*cos(q1L))/81129638414606681695789005144064 - (43889380989894851923989405068805*sin(q1L))/81129638414606681695789005144064 + 63594381400292563045725890951477/664613997892457936451903530140172288))/9007199254740992 + (7514214926474921*cos(q3L)*((7514214926474921*cos(q2L)*((6283307137322267*cos(q1L))/9007199254740992 - (4872700232219253*sin(q1L))/9007199254740992))/36893488147419103232 - (76229820211215127867025072518845*cos(q2L))/162259276829213363391578010288128 + sin(q2L)*((4872700232219253*cos(q1L))/9007199254740992 + (6283307137322267*sin(q1L))/9007199254740992)))/36893488147419103232 - sin(q3L)*((76229820211215127867025072518845*sin(q2L))/162259276829213363391578010288128 + cos(q2L)*((4872700232219253*cos(q1L))/9007199254740992 + (6283307137322267*sin(q1L))/9007199254740992) - (7514214926474921*sin(q2L)*((6283307137322267*cos(q1L))/9007199254740992 - (4872700232219253*sin(q1L))/9007199254740992))/36893488147419103232)) - (7514214926474921*sin(q4L)*((9007199067919185*sin(q3L)*((56594998190739085871744456992395*cos(q1L))/81129638414606681695789005144064 - (43889380989894851923989405068805*sin(q1L))/81129638414606681695789005144064 + 63594381400292563045725890951477/664613997892457936451903530140172288))/9007199254740992 + cos(q3L)*((76229820211215127867025072518845*sin(q2L))/162259276829213363391578010288128 + cos(q2L)*((4872700232219253*cos(q1L))/9007199254740992 + (6283307137322267*sin(q1L))/9007199254740992) - (7514214926474921*sin(q2L)*((6283307137322267*cos(q1L))/9007199254740992 - (4872700232219253*sin(q1L))/9007199254740992))/36893488147419103232) + (7514214926474921*sin(q3L)*((7514214926474921*cos(q2L)*((6283307137322267*cos(q1L))/9007199254740992 - (4872700232219253*sin(q1L))/9007199254740992))/36893488147419103232 - (76229820211215127867025072518845*cos(q2L))/162259276829213363391578010288128 + sin(q2L)*((4872700232219253*cos(q1L))/9007199254740992 + (6283307137322267*sin(q1L))/9007199254740992)))/36893488147419103232))/36893488147419103232)))/332306998946228968225951765070086144000 - (109198173955282063961996941994332957526645881091499469714283881779231664456243735535448036415347*cos(q3L)*((56594998190739085871744456992395*cos(q1L))/81129638414606681695789005144064 - (43889380989894851923989405068805*sin(q1L))/81129638414606681695789005144064 + 63594381400292563045725890951477/664613997892457936451903530140172288))/2607406049708142190423610481164004046145879543892398400814259775173608063697070983914748641280000 - (27*cos(q6L)*((9007199067919185*sin(q5L)*((2115063383689692319117831580025*cos(q3L)*((56594998190739085871744456992395*cos(q1L))/81129638414606681695789005144064 - (43889380989894851923989405068805*sin(q1L))/81129638414606681695789005144064 + 63594381400292563045725890951477/664613997892457936451903530140172288))/10384593717069655257060992658440192 + (81129635049124235038645691064225*sin(q3L)*((56594998190739085871744456992395*cos(q1L))/81129638414606681695789005144064 - (43889380989894851923989405068805*sin(q1L))/81129638414606681695789005144064 + 63594381400292563045725890951477/664613997892457936451903530140172288))/81129638414606681695789005144064 + (1764482024691522628700660907665*cos(q3L)*((7514214926474921*cos(q2L)*((6283307137322267*cos(q1L))/9007199254740992 - (4872700232219253*sin(q1L))/9007199254740992))/36893488147419103232 - (76229820211215127867025072518845*cos(q2L))/162259276829213363391578010288128 + sin(q2L)*((4872700232219253*cos(q1L))/9007199254740992 + (6283307137322267*sin(q1L))/9007199254740992)))/42535295865117307932921825928971026432 + (9007199067919185*cos(q3L)*((76229820211215127867025072518845*sin(q2L))/162259276829213363391578010288128 + cos(q2L)*((4872700232219253*cos(q1L))/9007199254740992 + (6283307137322267*sin(q1L))/9007199254740992) - (7514214926474921*sin(q2L)*((6283307137322267*cos(q1L))/9007199254740992 - (4872700232219253*sin(q1L))/9007199254740992))/36893488147419103232))/9007199254740992 + (67682029681889335677290557259385*sin(q3L)*((7514214926474921*cos(q2L)*((6283307137322267*cos(q1L))/9007199254740992 - (4872700232219253*sin(q1L))/9007199254740992))/36893488147419103232 - (76229820211215127867025072518845*cos(q2L))/162259276829213363391578010288128 + sin(q2L)*((4872700232219253*cos(q1L))/9007199254740992 + (6283307137322267*sin(q1L))/9007199254740992)))/332306998946228968225951765070086144 - (234819211581865*sin(q3L)*((76229820211215127867025072518845*sin(q2L))/162259276829213363391578010288128 + cos(q2L)*((4872700232219253*cos(q1L))/9007199254740992 + (6283307137322267*sin(q1L))/9007199254740992) - (7514214926474921*sin(q2L)*((6283307137322267*cos(q1L))/9007199254740992 - (4872700232219253*sin(q1L))/9007199254740992))/36893488147419103232))/1152921504606846976))/9007199254740992 + cos(q5L)*(((7514214926474921*cos(q4L))/36893488147419103232 + (4503599440548691*sin(q4L))/4503599627370496)*((9007199067919185*cos(q3L)*((56594998190739085871744456992395*cos(q1L))/81129638414606681695789005144064 - (43889380989894851923989405068805*sin(q1L))/81129638414606681695789005144064 + 63594381400292563045725890951477/664613997892457936451903530140172288))/9007199254740992 + (7514214926474921*cos(q3L)*((7514214926474921*cos(q2L)*((6283307137322267*cos(q1L))/9007199254740992 - (4872700232219253*sin(q1L))/9007199254740992))/36893488147419103232 - (76229820211215127867025072518845*cos(q2L))/162259276829213363391578010288128 + sin(q2L)*((4872700232219253*cos(q1L))/9007199254740992 + (6283307137322267*sin(q1L))/9007199254740992)))/36893488147419103232 - sin(q3L)*((76229820211215127867025072518845*sin(q2L))/162259276829213363391578010288128 + cos(q2L)*((4872700232219253*cos(q1L))/9007199254740992 + (6283307137322267*sin(q1L))/9007199254740992) - (7514214926474921*sin(q2L)*((6283307137322267*cos(q1L))/9007199254740992 - (4872700232219253*sin(q1L))/9007199254740992))/36893488147419103232)) - (7514214926474921*sin(q4L)*((9007199067919185*sin(q3L)*((56594998190739085871744456992395*cos(q1L))/81129638414606681695789005144064 - (43889380989894851923989405068805*sin(q1L))/81129638414606681695789005144064 + 63594381400292563045725890951477/664613997892457936451903530140172288))/9007199254740992 + cos(q3L)*((76229820211215127867025072518845*sin(q2L))/162259276829213363391578010288128 + cos(q2L)*((4872700232219253*cos(q1L))/9007199254740992 + (6283307137322267*sin(q1L))/9007199254740992) - (7514214926474921*sin(q2L)*((6283307137322267*cos(q1L))/9007199254740992 - (4872700232219253*sin(q1L))/9007199254740992))/36893488147419103232) + (7514214926474921*sin(q3L)*((7514214926474921*cos(q2L)*((6283307137322267*cos(q1L))/9007199254740992 - (4872700232219253*sin(q1L))/9007199254740992))/36893488147419103232 - (76229820211215127867025072518845*cos(q2L))/162259276829213363391578010288128 + sin(q2L)*((4872700232219253*cos(q1L))/9007199254740992 + (6283307137322267*sin(q1L))/9007199254740992)))/36893488147419103232))/36893488147419103232) - (7514214926474921*sin(q5L)*(((4503599440548691*cos(q4L))/4503599627370496 - (7514214926474921*sin(q4L))/36893488147419103232)*((9007199067919185*cos(q3L)*((56594998190739085871744456992395*cos(q1L))/81129638414606681695789005144064 - (43889380989894851923989405068805*sin(q1L))/81129638414606681695789005144064 + 63594381400292563045725890951477/664613997892457936451903530140172288))/9007199254740992 + (7514214926474921*cos(q3L)*((7514214926474921*cos(q2L)*((6283307137322267*cos(q1L))/9007199254740992 - (4872700232219253*sin(q1L))/9007199254740992))/36893488147419103232 - (76229820211215127867025072518845*cos(q2L))/162259276829213363391578010288128 + sin(q2L)*((4872700232219253*cos(q1L))/9007199254740992 + (6283307137322267*sin(q1L))/9007199254740992)))/36893488147419103232 - sin(q3L)*((76229820211215127867025072518845*sin(q2L))/162259276829213363391578010288128 + cos(q2L)*((4872700232219253*cos(q1L))/9007199254740992 + (6283307137322267*sin(q1L))/9007199254740992) - (7514214926474921*sin(q2L)*((6283307137322267*cos(q1L))/9007199254740992 - (4872700232219253*sin(q1L))/9007199254740992))/36893488147419103232)) - (7514214926474921*cos(q4L)*((9007199067919185*sin(q3L)*((56594998190739085871744456992395*cos(q1L))/81129638414606681695789005144064 - (43889380989894851923989405068805*sin(q1L))/81129638414606681695789005144064 + 63594381400292563045725890951477/664613997892457936451903530140172288))/9007199254740992 + cos(q3L)*((76229820211215127867025072518845*sin(q2L))/162259276829213363391578010288128 + cos(q2L)*((4872700232219253*cos(q1L))/9007199254740992 + (6283307137322267*sin(q1L))/9007199254740992) - (7514214926474921*sin(q2L)*((6283307137322267*cos(q1L))/9007199254740992 - (4872700232219253*sin(q1L))/9007199254740992))/36893488147419103232) + (7514214926474921*sin(q3L)*((7514214926474921*cos(q2L)*((6283307137322267*cos(q1L))/9007199254740992 - (4872700232219253*sin(q1L))/9007199254740992))/36893488147419103232 - (76229820211215127867025072518845*cos(q2L))/162259276829213363391578010288128 + sin(q2L)*((4872700232219253*cos(q1L))/9007199254740992 + (6283307137322267*sin(q1L))/9007199254740992)))/36893488147419103232))/36893488147419103232))/36893488147419103232))/1000 - (202883803014822867*sin(q6L)*((7514214926474921*cos(q5L)*(((4503599440548691*cos(q4L))/4503599627370496 - (7514214926474921*sin(q4L))/36893488147419103232)*((9007199067919185*cos(q3L)*((56594998190739085871744456992395*cos(q1L))/81129638414606681695789005144064 - (43889380989894851923989405068805*sin(q1L))/81129638414606681695789005144064 + 63594381400292563045725890951477/664613997892457936451903530140172288))/9007199254740992 + (7514214926474921*cos(q3L)*((7514214926474921*cos(q2L)*((6283307137322267*cos(q1L))/9007199254740992 - (4872700232219253*sin(q1L))/9007199254740992))/36893488147419103232 - (76229820211215127867025072518845*cos(q2L))/162259276829213363391578010288128 + sin(q2L)*((4872700232219253*cos(q1L))/9007199254740992 + (6283307137322267*sin(q1L))/9007199254740992)))/36893488147419103232 - sin(q3L)*((76229820211215127867025072518845*sin(q2L))/162259276829213363391578010288128 + cos(q2L)*((4872700232219253*cos(q1L))/9007199254740992 + (6283307137322267*sin(q1L))/9007199254740992) - (7514214926474921*sin(q2L)*((6283307137322267*cos(q1L))/9007199254740992 - (4872700232219253*sin(q1L))/9007199254740992))/36893488147419103232)) - (7514214926474921*cos(q4L)*((9007199067919185*sin(q3L)*((56594998190739085871744456992395*cos(q1L))/81129638414606681695789005144064 - (43889380989894851923989405068805*sin(q1L))/81129638414606681695789005144064 + 63594381400292563045725890951477/664613997892457936451903530140172288))/9007199254740992 + cos(q3L)*((76229820211215127867025072518845*sin(q2L))/162259276829213363391578010288128 + cos(q2L)*((4872700232219253*cos(q1L))/9007199254740992 + (6283307137322267*sin(q1L))/9007199254740992) - (7514214926474921*sin(q2L)*((6283307137322267*cos(q1L))/9007199254740992 - (4872700232219253*sin(q1L))/9007199254740992))/36893488147419103232) + (7514214926474921*sin(q3L)*((7514214926474921*cos(q2L)*((6283307137322267*cos(q1L))/9007199254740992 - (4872700232219253*sin(q1L))/9007199254740992))/36893488147419103232 - (76229820211215127867025072518845*cos(q2L))/162259276829213363391578010288128 + sin(q2L)*((4872700232219253*cos(q1L))/9007199254740992 + (6283307137322267*sin(q1L))/9007199254740992)))/36893488147419103232))/36893488147419103232))/36893488147419103232 - (9007199067919185*cos(q5L)*((2115063383689692319117831580025*cos(q3L)*((56594998190739085871744456992395*cos(q1L))/81129638414606681695789005144064 - (43889380989894851923989405068805*sin(q1L))/81129638414606681695789005144064 + 63594381400292563045725890951477/664613997892457936451903530140172288))/10384593717069655257060992658440192 + (81129635049124235038645691064225*sin(q3L)*((56594998190739085871744456992395*cos(q1L))/81129638414606681695789005144064 - (43889380989894851923989405068805*sin(q1L))/81129638414606681695789005144064 + 63594381400292563045725890951477/664613997892457936451903530140172288))/81129638414606681695789005144064 + (1764482024691522628700660907665*cos(q3L)*((7514214926474921*cos(q2L)*((6283307137322267*cos(q1L))/9007199254740992 - (4872700232219253*sin(q1L))/9007199254740992))/36893488147419103232 - (76229820211215127867025072518845*cos(q2L))/162259276829213363391578010288128 + sin(q2L)*((4872700232219253*cos(q1L))/9007199254740992 + (6283307137322267*sin(q1L))/9007199254740992)))/42535295865117307932921825928971026432 + (9007199067919185*cos(q3L)*((76229820211215127867025072518845*sin(q2L))/162259276829213363391578010288128 + cos(q2L)*((4872700232219253*cos(q1L))/9007199254740992 + (6283307137322267*sin(q1L))/9007199254740992) - (7514214926474921*sin(q2L)*((6283307137322267*cos(q1L))/9007199254740992 - (4872700232219253*sin(q1L))/9007199254740992))/36893488147419103232))/9007199254740992 + (67682029681889335677290557259385*sin(q3L)*((7514214926474921*cos(q2L)*((6283307137322267*cos(q1L))/9007199254740992 - (4872700232219253*sin(q1L))/9007199254740992))/36893488147419103232 - (76229820211215127867025072518845*cos(q2L))/162259276829213363391578010288128 + sin(q2L)*((4872700232219253*cos(q1L))/9007199254740992 + (6283307137322267*sin(q1L))/9007199254740992)))/332306998946228968225951765070086144 - (234819211581865*sin(q3L)*((76229820211215127867025072518845*sin(q2L))/162259276829213363391578010288128 + cos(q2L)*((4872700232219253*cos(q1L))/9007199254740992 + (6283307137322267*sin(q1L))/9007199254740992) - (7514214926474921*sin(q2L)*((6283307137322267*cos(q1L))/9007199254740992 - (4872700232219253*sin(q1L))/9007199254740992))/36893488147419103232))/1152921504606846976))/9007199254740992 + sin(q5L)*(((7514214926474921*cos(q4L))/36893488147419103232 + (4503599440548691*sin(q4L))/4503599627370496)*((9007199067919185*cos(q3L)*((56594998190739085871744456992395*cos(q1L))/81129638414606681695789005144064 - (43889380989894851923989405068805*sin(q1L))/81129638414606681695789005144064 + 63594381400292563045725890951477/664613997892457936451903530140172288))/9007199254740992 + (7514214926474921*cos(q3L)*((7514214926474921*cos(q2L)*((6283307137322267*cos(q1L))/9007199254740992 - (4872700232219253*sin(q1L))/9007199254740992))/36893488147419103232 - (76229820211215127867025072518845*cos(q2L))/162259276829213363391578010288128 + sin(q2L)*((4872700232219253*cos(q1L))/9007199254740992 + (6283307137322267*sin(q1L))/9007199254740992)))/36893488147419103232 - sin(q3L)*((76229820211215127867025072518845*sin(q2L))/162259276829213363391578010288128 + cos(q2L)*((4872700232219253*cos(q1L))/9007199254740992 + (6283307137322267*sin(q1L))/9007199254740992) - (7514214926474921*sin(q2L)*((6283307137322267*cos(q1L))/9007199254740992 - (4872700232219253*sin(q1L))/9007199254740992))/36893488147419103232)) - (7514214926474921*sin(q4L)*((9007199067919185*sin(q3L)*((56594998190739085871744456992395*cos(q1L))/81129638414606681695789005144064 - (43889380989894851923989405068805*sin(q1L))/81129638414606681695789005144064 + 63594381400292563045725890951477/664613997892457936451903530140172288))/9007199254740992 + cos(q3L)*((76229820211215127867025072518845*sin(q2L))/162259276829213363391578010288128 + cos(q2L)*((4872700232219253*cos(q1L))/9007199254740992 + (6283307137322267*sin(q1L))/9007199254740992) - (7514214926474921*sin(q2L)*((6283307137322267*cos(q1L))/9007199254740992 - (4872700232219253*sin(q1L))/9007199254740992))/36893488147419103232) + (7514214926474921*sin(q3L)*((7514214926474921*cos(q2L)*((6283307137322267*cos(q1L))/9007199254740992 - (4872700232219253*sin(q1L))/9007199254740992))/36893488147419103232 - (76229820211215127867025072518845*cos(q2L))/162259276829213363391578010288128 + sin(q2L)*((4872700232219253*cos(q1L))/9007199254740992 + (6283307137322267*sin(q1L))/9007199254740992)))/36893488147419103232))/36893488147419103232)))/36893488147419103232000 - (584133382113593486367040631332731*cos(q6L)*((15893040848161638993908057577265778144967053025*cos(q3L)*((56594998190739085871744456992395*cos(q1L))/81129638414606681695789005144064 - (43889380989894851923989405068805*sin(q1L))/81129638414606681695789005144064 + 63594381400292563045725890951477/664613997892457936451903530140172288))/383123885216472214589586756787577295904684780545900544 + (609625514665592237562888769449172969868262801225*sin(q3L)*((56594998190739085871744456992395*cos(q1L))/81129638414606681695789005144064 - (43889380989894851923989405068805*sin(q1L))/81129638414606681695789005144064 + 63594381400292563045725890951477/664613997892457936451903530140172288))/2993155353253689176481146537402947624255349848014848 + (9007199067919185*((4503599440548691*cos(q4L))/4503599627370496 - (7514214926474921*sin(q4L))/36893488147419103232)*((9007199067919185*cos(q3L)*((56594998190739085871744456992395*cos(q1L))/81129638414606681695789005144064 - (43889380989894851923989405068805*sin(q1L))/81129638414606681695789005144064 + 63594381400292563045725890951477/664613997892457936451903530140172288))/9007199254740992 + (7514214926474921*cos(q3L)*((7514214926474921*cos(q2L)*((6283307137322267*cos(q1L))/9007199254740992 - (4872700232219253*sin(q1L))/9007199254740992))/36893488147419103232 - (76229820211215127867025072518845*cos(q2L))/162259276829213363391578010288128 + sin(q2L)*((4872700232219253*cos(q1L))/9007199254740992 + (6283307137322267*sin(q1L))/9007199254740992)))/36893488147419103232 - sin(q3L)*((76229820211215127867025072518845*sin(q2L))/162259276829213363391578010288128 + cos(q2L)*((4872700232219253*cos(q1L))/9007199254740992 + (6283307137322267*sin(q1L))/9007199254740992) - (7514214926474921*sin(q2L)*((6283307137322267*cos(q1L))/9007199254740992 - (4872700232219253*sin(q1L))/9007199254740992))/36893488147419103232)))/9007199254740992 + (13258697167433729449897784796786197386719169465*cos(q3L)*((7514214926474921*cos(q2L)*((6283307137322267*cos(q1L))/9007199254740992 - (4872700232219253*sin(q1L))/9007199254740992))/36893488147419103232 - (76229820211215127867025072518845*cos(q2L))/162259276829213363391578010288128 + sin(q2L)*((4872700232219253*cos(q1L))/9007199254740992 + (6283307137322267*sin(q1L))/9007199254740992)))/1569275433846670190958947355801916604025588861116008628224 + (67682029681889335677290557259385*cos(q3L)*((76229820211215127867025072518845*sin(q2L))/162259276829213363391578010288128 + cos(q2L)*((4872700232219253*cos(q1L))/9007199254740992 + (6283307137322267*sin(q1L))/9007199254740992) - (7514214926474921*sin(q2L)*((6283307137322267*cos(q1L))/9007199254740992 - (4872700232219253*sin(q1L))/9007199254740992))/36893488147419103232))/332306998946228968225951765070086144 + (508577317689771495245073589786522929324694383585*sin(q3L)*((7514214926474921*cos(q2L)*((6283307137322267*cos(q1L))/9007199254740992 - (4872700232219253*sin(q1L))/9007199254740992))/36893488147419103232 - (76229820211215127867025072518845*cos(q2L))/162259276829213363391578010288128 + sin(q2L)*((4872700232219253*cos(q1L))/9007199254740992 + (6283307137322267*sin(q1L))/9007199254740992)))/12259964326927110866866776217202473468949912977468817408 - (1764482024691522628700660907665*sin(q3L)*((76229820211215127867025072518845*sin(q2L))/162259276829213363391578010288128 + cos(q2L)*((4872700232219253*cos(q1L))/9007199254740992 + (6283307137322267*sin(q1L))/9007199254740992) - (7514214926474921*sin(q2L)*((6283307137322267*cos(q1L))/9007199254740992 - (4872700232219253*sin(q1L))/9007199254740992))/36893488147419103232))/42535295865117307932921825928971026432 - (67682029681889335677290557259385*cos(q4L)*((9007199067919185*sin(q3L)*((56594998190739085871744456992395*cos(q1L))/81129638414606681695789005144064 - (43889380989894851923989405068805*sin(q1L))/81129638414606681695789005144064 + 63594381400292563045725890951477/664613997892457936451903530140172288))/9007199254740992 + cos(q3L)*((76229820211215127867025072518845*sin(q2L))/162259276829213363391578010288128 + cos(q2L)*((4872700232219253*cos(q1L))/9007199254740992 + (6283307137322267*sin(q1L))/9007199254740992) - (7514214926474921*sin(q2L)*((6283307137322267*cos(q1L))/9007199254740992 - (4872700232219253*sin(q1L))/9007199254740992))/36893488147419103232) + (7514214926474921*sin(q3L)*((7514214926474921*cos(q2L)*((6283307137322267*cos(q1L))/9007199254740992 - (4872700232219253*sin(q1L))/9007199254740992))/36893488147419103232 - (76229820211215127867025072518845*cos(q2L))/162259276829213363391578010288128 + sin(q2L)*((4872700232219253*cos(q1L))/9007199254740992 + (6283307137322267*sin(q1L))/9007199254740992)))/36893488147419103232))/332306998946228968225951765070086144))/16225927682921336339157801028812800 - (170695144106365826517608855445768431563113584343*cos(q5L)*((2115063383689692319117831580025*cos(q3L)*((56594998190739085871744456992395*cos(q1L))/81129638414606681695789005144064 - (43889380989894851923989405068805*sin(q1L))/81129638414606681695789005144064 + 63594381400292563045725890951477/664613997892457936451903530140172288))/10384593717069655257060992658440192 + (81129635049124235038645691064225*sin(q3L)*((56594998190739085871744456992395*cos(q1L))/81129638414606681695789005144064 - (43889380989894851923989405068805*sin(q1L))/81129638414606681695789005144064 + 63594381400292563045725890951477/664613997892457936451903530140172288))/81129638414606681695789005144064 + (1764482024691522628700660907665*cos(q3L)*((7514214926474921*cos(q2L)*((6283307137322267*cos(q1L))/9007199254740992 - (4872700232219253*sin(q1L))/9007199254740992))/36893488147419103232 - (76229820211215127867025072518845*cos(q2L))/162259276829213363391578010288128 + sin(q2L)*((4872700232219253*cos(q1L))/9007199254740992 + (6283307137322267*sin(q1L))/9007199254740992)))/42535295865117307932921825928971026432 + (9007199067919185*cos(q3L)*((76229820211215127867025072518845*sin(q2L))/162259276829213363391578010288128 + cos(q2L)*((4872700232219253*cos(q1L))/9007199254740992 + (6283307137322267*sin(q1L))/9007199254740992) - (7514214926474921*sin(q2L)*((6283307137322267*cos(q1L))/9007199254740992 - (4872700232219253*sin(q1L))/9007199254740992))/36893488147419103232))/9007199254740992 + (67682029681889335677290557259385*sin(q3L)*((7514214926474921*cos(q2L)*((6283307137322267*cos(q1L))/9007199254740992 - (4872700232219253*sin(q1L))/9007199254740992))/36893488147419103232 - (76229820211215127867025072518845*cos(q2L))/162259276829213363391578010288128 + sin(q2L)*((4872700232219253*cos(q1L))/9007199254740992 + (6283307137322267*sin(q1L))/9007199254740992)))/332306998946228968225951765070086144 - (234819211581865*sin(q3L)*((76229820211215127867025072518845*sin(q2L))/162259276829213363391578010288128 + cos(q2L)*((4872700232219253*cos(q1L))/9007199254740992 + (6283307137322267*sin(q1L))/9007199254740992) - (7514214926474921*sin(q2L)*((6283307137322267*cos(q1L))/9007199254740992 - (4872700232219253*sin(q1L))/9007199254740992))/36893488147419103232))/1152921504606846976))/119726214130147567059245861496117904970213993920593920 + (324259171862923063*sin(q6L)*((9007199067919185*sin(q5L)*((2115063383689692319117831580025*cos(q3L)*((56594998190739085871744456992395*cos(q1L))/81129638414606681695789005144064 - (43889380989894851923989405068805*sin(q1L))/81129638414606681695789005144064 + 63594381400292563045725890951477/664613997892457936451903530140172288))/10384593717069655257060992658440192 + (81129635049124235038645691064225*sin(q3L)*((56594998190739085871744456992395*cos(q1L))/81129638414606681695789005144064 - (43889380989894851923989405068805*sin(q1L))/81129638414606681695789005144064 + 63594381400292563045725890951477/664613997892457936451903530140172288))/81129638414606681695789005144064 + (1764482024691522628700660907665*cos(q3L)*((7514214926474921*cos(q2L)*((6283307137322267*cos(q1L))/9007199254740992 - (4872700232219253*sin(q1L))/9007199254740992))/36893488147419103232 - (76229820211215127867025072518845*cos(q2L))/162259276829213363391578010288128 + sin(q2L)*((4872700232219253*cos(q1L))/9007199254740992 + (6283307137322267*sin(q1L))/9007199254740992)))/42535295865117307932921825928971026432 + (9007199067919185*cos(q3L)*((76229820211215127867025072518845*sin(q2L))/162259276829213363391578010288128 + cos(q2L)*((4872700232219253*cos(q1L))/9007199254740992 + (6283307137322267*sin(q1L))/9007199254740992) - (7514214926474921*sin(q2L)*((6283307137322267*cos(q1L))/9007199254740992 - (4872700232219253*sin(q1L))/9007199254740992))/36893488147419103232))/9007199254740992 + (67682029681889335677290557259385*sin(q3L)*((7514214926474921*cos(q2L)*((6283307137322267*cos(q1L))/9007199254740992 - (4872700232219253*sin(q1L))/9007199254740992))/36893488147419103232 - (76229820211215127867025072518845*cos(q2L))/162259276829213363391578010288128 + sin(q2L)*((4872700232219253*cos(q1L))/9007199254740992 + (6283307137322267*sin(q1L))/9007199254740992)))/332306998946228968225951765070086144 - (234819211581865*sin(q3L)*((76229820211215127867025072518845*sin(q2L))/162259276829213363391578010288128 + cos(q2L)*((4872700232219253*cos(q1L))/9007199254740992 + (6283307137322267*sin(q1L))/9007199254740992) - (7514214926474921*sin(q2L)*((6283307137322267*cos(q1L))/9007199254740992 - (4872700232219253*sin(q1L))/9007199254740992))/36893488147419103232))/1152921504606846976))/9007199254740992 + cos(q5L)*(((7514214926474921*cos(q4L))/36893488147419103232 + (4503599440548691*sin(q4L))/4503599627370496)*((9007199067919185*cos(q3L)*((56594998190739085871744456992395*cos(q1L))/81129638414606681695789005144064 - (43889380989894851923989405068805*sin(q1L))/81129638414606681695789005144064 + 63594381400292563045725890951477/664613997892457936451903530140172288))/9007199254740992 + (7514214926474921*cos(q3L)*((7514214926474921*cos(q2L)*((6283307137322267*cos(q1L))/9007199254740992 - (4872700232219253*sin(q1L))/9007199254740992))/36893488147419103232 - (76229820211215127867025072518845*cos(q2L))/162259276829213363391578010288128 + sin(q2L)*((4872700232219253*cos(q1L))/9007199254740992 + (6283307137322267*sin(q1L))/9007199254740992)))/36893488147419103232 - sin(q3L)*((76229820211215127867025072518845*sin(q2L))/162259276829213363391578010288128 + cos(q2L)*((4872700232219253*cos(q1L))/9007199254740992 + (6283307137322267*sin(q1L))/9007199254740992) - (7514214926474921*sin(q2L)*((6283307137322267*cos(q1L))/9007199254740992 - (4872700232219253*sin(q1L))/9007199254740992))/36893488147419103232)) - (7514214926474921*sin(q4L)*((9007199067919185*sin(q3L)*((56594998190739085871744456992395*cos(q1L))/81129638414606681695789005144064 - (43889380989894851923989405068805*sin(q1L))/81129638414606681695789005144064 + 63594381400292563045725890951477/664613997892457936451903530140172288))/9007199254740992 + cos(q3L)*((76229820211215127867025072518845*sin(q2L))/162259276829213363391578010288128 + cos(q2L)*((4872700232219253*cos(q1L))/9007199254740992 + (6283307137322267*sin(q1L))/9007199254740992) - (7514214926474921*sin(q2L)*((6283307137322267*cos(q1L))/9007199254740992 - (4872700232219253*sin(q1L))/9007199254740992))/36893488147419103232) + (7514214926474921*sin(q3L)*((7514214926474921*cos(q2L)*((6283307137322267*cos(q1L))/9007199254740992 - (4872700232219253*sin(q1L))/9007199254740992))/36893488147419103232 - (76229820211215127867025072518845*cos(q2L))/162259276829213363391578010288128 + sin(q2L)*((4872700232219253*cos(q1L))/9007199254740992 + (6283307137322267*sin(q1L))/9007199254740992)))/36893488147419103232))/36893488147419103232) - (7514214926474921*sin(q5L)*(((4503599440548691*cos(q4L))/4503599627370496 - (7514214926474921*sin(q4L))/36893488147419103232)*((9007199067919185*cos(q3L)*((56594998190739085871744456992395*cos(q1L))/81129638414606681695789005144064 - (43889380989894851923989405068805*sin(q1L))/81129638414606681695789005144064 + 63594381400292563045725890951477/664613997892457936451903530140172288))/9007199254740992 + (7514214926474921*cos(q3L)*((7514214926474921*cos(q2L)*((6283307137322267*cos(q1L))/9007199254740992 - (4872700232219253*sin(q1L))/9007199254740992))/36893488147419103232 - (76229820211215127867025072518845*cos(q2L))/162259276829213363391578010288128 + sin(q2L)*((4872700232219253*cos(q1L))/9007199254740992 + (6283307137322267*sin(q1L))/9007199254740992)))/36893488147419103232 - sin(q3L)*((76229820211215127867025072518845*sin(q2L))/162259276829213363391578010288128 + cos(q2L)*((4872700232219253*cos(q1L))/9007199254740992 + (6283307137322267*sin(q1L))/9007199254740992) - (7514214926474921*sin(q2L)*((6283307137322267*cos(q1L))/9007199254740992 - (4872700232219253*sin(q1L))/9007199254740992))/36893488147419103232)) - (7514214926474921*cos(q4L)*((9007199067919185*sin(q3L)*((56594998190739085871744456992395*cos(q1L))/81129638414606681695789005144064 - (43889380989894851923989405068805*sin(q1L))/81129638414606681695789005144064 + 63594381400292563045725890951477/664613997892457936451903530140172288))/9007199254740992 + cos(q3L)*((76229820211215127867025072518845*sin(q2L))/162259276829213363391578010288128 + cos(q2L)*((4872700232219253*cos(q1L))/9007199254740992 + (6283307137322267*sin(q1L))/9007199254740992) - (7514214926474921*sin(q2L)*((6283307137322267*cos(q1L))/9007199254740992 - (4872700232219253*sin(q1L))/9007199254740992))/36893488147419103232) + (7514214926474921*sin(q3L)*((7514214926474921*cos(q2L)*((6283307137322267*cos(q1L))/9007199254740992 - (4872700232219253*sin(q1L))/9007199254740992))/36893488147419103232 - (76229820211215127867025072518845*cos(q2L))/162259276829213363391578010288128 + sin(q2L)*((4872700232219253*cos(q1L))/9007199254740992 + (6283307137322267*sin(q1L))/9007199254740992)))/36893488147419103232))/36893488147419103232))/36893488147419103232))/9007199254740992000 - (48638874966763599*sin(q6L)*((15893040848161638993908057577265778144967053025*cos(q3L)*((56594998190739085871744456992395*cos(q1L))/81129638414606681695789005144064 - (43889380989894851923989405068805*sin(q1L))/81129638414606681695789005144064 + 63594381400292563045725890951477/664613997892457936451903530140172288))/383123885216472214589586756787577295904684780545900544 + (609625514665592237562888769449172969868262801225*sin(q3L)*((56594998190739085871744456992395*cos(q1L))/81129638414606681695789005144064 - (43889380989894851923989405068805*sin(q1L))/81129638414606681695789005144064 + 63594381400292563045725890951477/664613997892457936451903530140172288))/2993155353253689176481146537402947624255349848014848 + (9007199067919185*((4503599440548691*cos(q4L))/4503599627370496 - (7514214926474921*sin(q4L))/36893488147419103232)*((9007199067919185*cos(q3L)*((56594998190739085871744456992395*cos(q1L))/81129638414606681695789005144064 - (43889380989894851923989405068805*sin(q1L))/81129638414606681695789005144064 + 63594381400292563045725890951477/664613997892457936451903530140172288))/9007199254740992 + (7514214926474921*cos(q3L)*((7514214926474921*cos(q2L)*((6283307137322267*cos(q1L))/9007199254740992 - (4872700232219253*sin(q1L))/9007199254740992))/36893488147419103232 - (76229820211215127867025072518845*cos(q2L))/162259276829213363391578010288128 + sin(q2L)*((4872700232219253*cos(q1L))/9007199254740992 + (6283307137322267*sin(q1L))/9007199254740992)))/36893488147419103232 - sin(q3L)*((76229820211215127867025072518845*sin(q2L))/162259276829213363391578010288128 + cos(q2L)*((4872700232219253*cos(q1L))/9007199254740992 + (6283307137322267*sin(q1L))/9007199254740992) - (7514214926474921*sin(q2L)*((6283307137322267*cos(q1L))/9007199254740992 - (4872700232219253*sin(q1L))/9007199254740992))/36893488147419103232)))/9007199254740992 + (13258697167433729449897784796786197386719169465*cos(q3L)*((7514214926474921*cos(q2L)*((6283307137322267*cos(q1L))/9007199254740992 - (4872700232219253*sin(q1L))/9007199254740992))/36893488147419103232 - (76229820211215127867025072518845*cos(q2L))/162259276829213363391578010288128 + sin(q2L)*((4872700232219253*cos(q1L))/9007199254740992 + (6283307137322267*sin(q1L))/9007199254740992)))/1569275433846670190958947355801916604025588861116008628224 + (67682029681889335677290557259385*cos(q3L)*((76229820211215127867025072518845*sin(q2L))/162259276829213363391578010288128 + cos(q2L)*((4872700232219253*cos(q1L))/9007199254740992 + (6283307137322267*sin(q1L))/9007199254740992) - (7514214926474921*sin(q2L)*((6283307137322267*cos(q1L))/9007199254740992 - (4872700232219253*sin(q1L))/9007199254740992))/36893488147419103232))/332306998946228968225951765070086144 + (508577317689771495245073589786522929324694383585*sin(q3L)*((7514214926474921*cos(q2L)*((6283307137322267*cos(q1L))/9007199254740992 - (4872700232219253*sin(q1L))/9007199254740992))/36893488147419103232 - (76229820211215127867025072518845*cos(q2L))/162259276829213363391578010288128 + sin(q2L)*((4872700232219253*cos(q1L))/9007199254740992 + (6283307137322267*sin(q1L))/9007199254740992)))/12259964326927110866866776217202473468949912977468817408 - (1764482024691522628700660907665*sin(q3L)*((76229820211215127867025072518845*sin(q2L))/162259276829213363391578010288128 + cos(q2L)*((4872700232219253*cos(q1L))/9007199254740992 + (6283307137322267*sin(q1L))/9007199254740992) - (7514214926474921*sin(q2L)*((6283307137322267*cos(q1L))/9007199254740992 - (4872700232219253*sin(q1L))/9007199254740992))/36893488147419103232))/42535295865117307932921825928971026432 - (67682029681889335677290557259385*cos(q4L)*((9007199067919185*sin(q3L)*((56594998190739085871744456992395*cos(q1L))/81129638414606681695789005144064 - (43889380989894851923989405068805*sin(q1L))/81129638414606681695789005144064 + 63594381400292563045725890951477/664613997892457936451903530140172288))/9007199254740992 + cos(q3L)*((76229820211215127867025072518845*sin(q2L))/162259276829213363391578010288128 + cos(q2L)*((4872700232219253*cos(q1L))/9007199254740992 + (6283307137322267*sin(q1L))/9007199254740992) - (7514214926474921*sin(q2L)*((6283307137322267*cos(q1L))/9007199254740992 - (4872700232219253*sin(q1L))/9007199254740992))/36893488147419103232) + (7514214926474921*sin(q3L)*((7514214926474921*cos(q2L)*((6283307137322267*cos(q1L))/9007199254740992 - (4872700232219253*sin(q1L))/9007199254740992))/36893488147419103232 - (76229820211215127867025072518845*cos(q2L))/162259276829213363391578010288128 + sin(q2L)*((4872700232219253*cos(q1L))/9007199254740992 + (6283307137322267*sin(q1L))/9007199254740992)))/36893488147419103232))/332306998946228968225951765070086144))/1801439850948198400 + (48638874966763599*sin(q5L)*((2115063383689692319117831580025*cos(q3L)*((56594998190739085871744456992395*cos(q1L))/81129638414606681695789005144064 - (43889380989894851923989405068805*sin(q1L))/81129638414606681695789005144064 + 63594381400292563045725890951477/664613997892457936451903530140172288))/10384593717069655257060992658440192 + (81129635049124235038645691064225*sin(q3L)*((56594998190739085871744456992395*cos(q1L))/81129638414606681695789005144064 - (43889380989894851923989405068805*sin(q1L))/81129638414606681695789005144064 + 63594381400292563045725890951477/664613997892457936451903530140172288))/81129638414606681695789005144064 + (1764482024691522628700660907665*cos(q3L)*((7514214926474921*cos(q2L)*((6283307137322267*cos(q1L))/9007199254740992 - (4872700232219253*sin(q1L))/9007199254740992))/36893488147419103232 - (76229820211215127867025072518845*cos(q2L))/162259276829213363391578010288128 + sin(q2L)*((4872700232219253*cos(q1L))/9007199254740992 + (6283307137322267*sin(q1L))/9007199254740992)))/42535295865117307932921825928971026432 + (9007199067919185*cos(q3L)*((76229820211215127867025072518845*sin(q2L))/162259276829213363391578010288128 + cos(q2L)*((4872700232219253*cos(q1L))/9007199254740992 + (6283307137322267*sin(q1L))/9007199254740992) - (7514214926474921*sin(q2L)*((6283307137322267*cos(q1L))/9007199254740992 - (4872700232219253*sin(q1L))/9007199254740992))/36893488147419103232))/9007199254740992 + (67682029681889335677290557259385*sin(q3L)*((7514214926474921*cos(q2L)*((6283307137322267*cos(q1L))/9007199254740992 - (4872700232219253*sin(q1L))/9007199254740992))/36893488147419103232 - (76229820211215127867025072518845*cos(q2L))/162259276829213363391578010288128 + sin(q2L)*((4872700232219253*cos(q1L))/9007199254740992 + (6283307137322267*sin(q1L))/9007199254740992)))/332306998946228968225951765070086144 - (234819211581865*sin(q3L)*((76229820211215127867025072518845*sin(q2L))/162259276829213363391578010288128 + cos(q2L)*((4872700232219253*cos(q1L))/9007199254740992 + (6283307137322267*sin(q1L))/9007199254740992) - (7514214926474921*sin(q2L)*((6283307137322267*cos(q1L))/9007199254740992 - (4872700232219253*sin(q1L))/9007199254740992))/36893488147419103232))/1152921504606846976))/1801439850948198400 + (610321541873521657855151997354401418608858870661075444886782706002880706727*cos(q4L)*((9007199067919185*sin(q3L)*((56594998190739085871744456992395*cos(q1L))/81129638414606681695789005144064 - (43889380989894851923989405068805*sin(q1L))/81129638414606681695789005144064 + 63594381400292563045725890951477/664613997892457936451903530140172288))/9007199254740992 + cos(q3L)*((76229820211215127867025072518845*sin(q2L))/162259276829213363391578010288128 + cos(q2L)*((4872700232219253*cos(q1L))/9007199254740992 + (6283307137322267*sin(q1L))/9007199254740992) - (7514214926474921*sin(q2L)*((6283307137322267*cos(q1L))/9007199254740992 - (4872700232219253*sin(q1L))/9007199254740992))/36893488147419103232) + (7514214926474921*sin(q3L)*((7514214926474921*cos(q2L)*((6283307137322267*cos(q1L))/9007199254740992 - (4872700232219253*sin(q1L))/9007199254740992))/36893488147419103232 - (76229820211215127867025072518845*cos(q2L))/162259276829213363391578010288128 + sin(q2L)*((4872700232219253*cos(q1L))/9007199254740992 + (6283307137322267*sin(q1L))/9007199254740992)))/36893488147419103232))/11307821214581659709333104004754678501295896940003961331978279688272766566400000 + (608651409044468601*sin(q4L)*((9007199067919185*sin(q3L)*((56594998190739085871744456992395*cos(q1L))/81129638414606681695789005144064 - (43889380989894851923989405068805*sin(q1L))/81129638414606681695789005144064 + 63594381400292563045725890951477/664613997892457936451903530140172288))/9007199254740992 + cos(q3L)*((76229820211215127867025072518845*sin(q2L))/162259276829213363391578010288128 + cos(q2L)*((4872700232219253*cos(q1L))/9007199254740992 + (6283307137322267*sin(q1L))/9007199254740992) - (7514214926474921*sin(q2L)*((6283307137322267*cos(q1L))/9007199254740992 - (4872700232219253*sin(q1L))/9007199254740992))/36893488147419103232) + (7514214926474921*sin(q3L)*((7514214926474921*cos(q2L)*((6283307137322267*cos(q1L))/9007199254740992 - (4872700232219253*sin(q1L))/9007199254740992))/36893488147419103232 - (76229820211215127867025072518845*cos(q2L))/162259276829213363391578010288128 + sin(q2L)*((4872700232219253*cos(q1L))/9007199254740992 + (6283307137322267*sin(q1L))/9007199254740992)))/36893488147419103232))/73786976294838206464000 + (712008244765680093343103025701132101054572137019*cos(q5L)*(((4503599440548691*cos(q4L))/4503599627370496 - (7514214926474921*sin(q4L))/36893488147419103232)*((9007199067919185*cos(q3L)*((56594998190739085871744456992395*cos(q1L))/81129638414606681695789005144064 - (43889380989894851923989405068805*sin(q1L))/81129638414606681695789005144064 + 63594381400292563045725890951477/664613997892457936451903530140172288))/9007199254740992 + (7514214926474921*cos(q3L)*((7514214926474921*cos(q2L)*((6283307137322267*cos(q1L))/9007199254740992 - (4872700232219253*sin(q1L))/9007199254740992))/36893488147419103232 - (76229820211215127867025072518845*cos(q2L))/162259276829213363391578010288128 + sin(q2L)*((4872700232219253*cos(q1L))/9007199254740992 + (6283307137322267*sin(q1L))/9007199254740992)))/36893488147419103232 - sin(q3L)*((76229820211215127867025072518845*sin(q2L))/162259276829213363391578010288128 + cos(q2L)*((4872700232219253*cos(q1L))/9007199254740992 + (6283307137322267*sin(q1L))/9007199254740992) - (7514214926474921*sin(q2L)*((6283307137322267*cos(q1L))/9007199254740992 - (4872700232219253*sin(q1L))/9007199254740992))/36893488147419103232)) - (7514214926474921*cos(q4L)*((9007199067919185*sin(q3L)*((56594998190739085871744456992395*cos(q1L))/81129638414606681695789005144064 - (43889380989894851923989405068805*sin(q1L))/81129638414606681695789005144064 + 63594381400292563045725890951477/664613997892457936451903530140172288))/9007199254740992 + cos(q3L)*((76229820211215127867025072518845*sin(q2L))/162259276829213363391578010288128 + cos(q2L)*((4872700232219253*cos(q1L))/9007199254740992 + (6283307137322267*sin(q1L))/9007199254740992) - (7514214926474921*sin(q2L)*((6283307137322267*cos(q1L))/9007199254740992 - (4872700232219253*sin(q1L))/9007199254740992))/36893488147419103232) + (7514214926474921*sin(q3L)*((7514214926474921*cos(q2L)*((6283307137322267*cos(q1L))/9007199254740992 - 